simulink library "vmc"  (R2021b)
settings: Solver=VariableStepAuto  StartTime=0.0  StopTime=10.0  RelTol=1e-3
undefined symbols (not defined in the file): AVMC_ACCDeltaTqGradeGn_X_deg, AVMC_ACCDeltaTqIGain4OVRD_X_kph, AVMC_ACCDeltaTqIGain4OVRD_Y_mps2, AVMC_ACCDeltaTqIGain_X_kph, AVMC_ACCDeltaTqIGain_Y_mps2, AVMC_ACCDeltaTqPGain_X_kph, AVMC_ACCDeltaTqPGain_Y_kph, AVMC_ACCGradeofst_X_G, AVMC_ACCGradeofst_Y_pct, AVMC_ACCLoSpdTqLoLim4JP_X_kph, AVMC_ACCLoSpdTqLoLim4JP_Y_deg, AVMC_ACCLoSpdTqLowerLim_X_kph, AVMC_ACCLoSpdTqLowerLim_Y_deg, AVMC_ACCReqAccelGain_X_mps2, AVMC_ACCReqAccelGain_Y_enum, AVMC_ADSPosGFBDeltaTq_X_kph, AVMC_ADSPosGFBDeltaTq_Y_mps2, AVMC_AggressJerkPCT4AT_X_kph, AVMC_AggressJerkPCT_X_kph, AVMC_AggressLimitPCT4AT_X_kph, AVMC_AggressLimitPCT_X_kph, AVMC_DECGradeofst_X_G, AVMC_DECGradeofst_Y_pct, AVMC_DISCDeltaTqIGain_X_kph, AVMC_DISCDeltaTqIGain_Y_mps2, AVMC_DISCDeltaTqPGain_X_kph, AVMC_DISCDeltaTqPGain_Y_kph, AVMC_EPSForceSelect_X_enum, AVMC_EPSForceSelect_Y_enum, AVMC_EPSForceSelectD21_X_enum, AVMC_EPSForceSelectD21_Y_enum, AVMC_ESCRegenOut_X_kph, AVMC_ESCRegenOut_Y_Deg, AVMC_ESCRegenOutEnSpd_X_Deg, AVMC_EstPitchSlopeTs_X_kph, AVMC_GradeCompFlt_X_kph, AVMC_GyroYBandLo_X_Gps, AVMC_HoldResTq_X_kph, AVMC_ISOAccLimit_X_mps, AVMC_ISODecLimit_X_mps, AVMC_ISOJerk_X_mps, AVMC_LatESCRegenOut_X_kph, AVMC_LatESCRegenOut_Y_Deg, AVMC_LongAccDeadZone_X_kph, AVMC_LongAccFiltTsforP2_X_Gps, AVMC_MCPresBaseTq_X_bar, AVMC_MSAPedalOvrd_X_kph, AVMC_MSASpdBand_X_kph, AVMC_MSATqDownEndTq_X_kph, AVMC_MSATqDownTime_X_kph, AVMC_NegZCHoldTq_X_kph, AVMC_OPDDisSlideRate_X_Deg, AVMC_OVRD2ActSR2FCMCMD_X_mps2, AVMC_PedalTqRWhlRatio_X_Nm, AVMC_PedalTqRWhlRatio_Y_gps, AVMC_PedalTqRWhlSlipGain_X_rat, AVMC_PedalTqRWhlSlipGain_Y_kph, AVMC_PedalTqRWhSTRGGain_X_deg, AVMC_PedalTqRWhSTRGGain_Y_kph, AVMC_PosZCHoldTq_X_kph ... (+593)
libraries: hcu_lib x143, simulink x96, tqr x4, $bdroot x1, simulink_extras x1
(part 2 of 17)

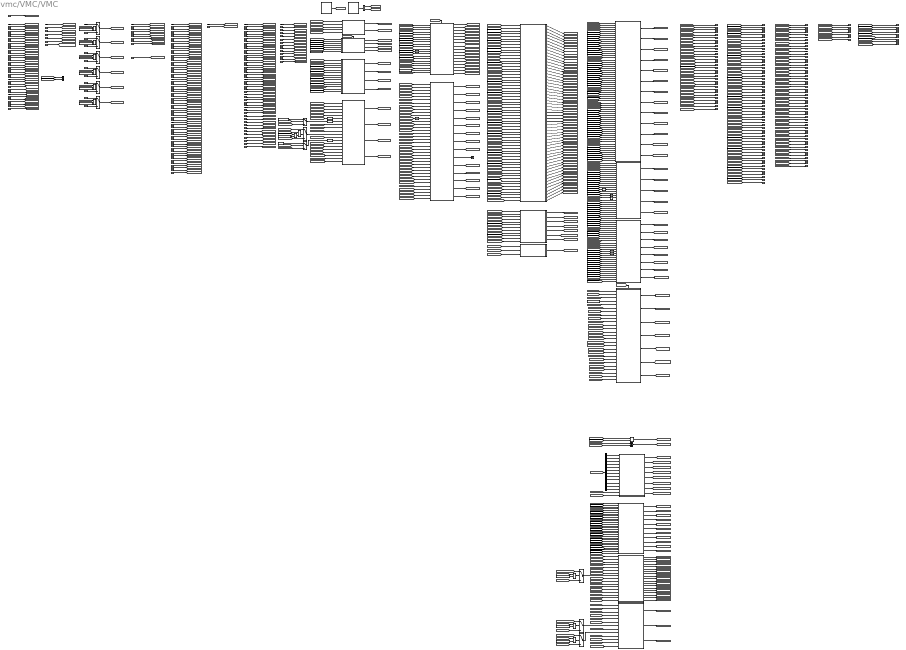
== system vmc/VMC/VMC ==
  note: CAN4
  note: For
      | DDM
      | 2025/02/18
  note: DSC
      | Test
      | Function
  note: SYS
  note: IMU
  note: SafetyControl
  note: ACC_CC_MSAWhlTq
  note: SpeedArbitration
  note: VMC_FCM1
  note: SPD2ACC
  note: PreConditionCheck
  note: KPH2MPH_SetSpeed
  note: CAN1
  note: CAN2
  note: CAN3
  note: DDM
  note: CAN6
  note: GPIO
  note: FD
  note: Phase1_Add Functions for VCU
  note: VMC SW Version:
      | CR-No. B14
      | Date: 2025/07/09
  note: AOICtrl
  task_time_s : Inport
  VINP_DriverSeatBeltCmd_flg : Inport  Port=2
  VINP_MeterIndVehSpeed_kph : Inport  Port=3
  VINP_BrkSwSta_flg : Inport  Port=4
  VINP_EPBSta_enum : Inport  Port=5
  VINP_ACCAvail_flg : Inport  Port=6
  VINP_AEBAvail_flg : Inport  Port=7
  VINP_ESCOFFStatus_enum : Inport  Port=8
  VINP_VehSpeed_kph : Inport  Port=9
  VINP_LFRawWhlSpeed_kph : Inport  Port=10
  VINP_LFRawWhlSpeedV_flg : Inport  Port=11
  VINP_RFRawWhlSpeed_kph : Inport  Port=12
  VINP_RFRawWhlSpeedV_flg : Inport  Port=13
  VINP_LRRawWhlSpeed_kph : Inport  Port=14
  VINP_LRRawWhlSpeedV_flg : Inport  Port=15
  VINP_RRRawWhlSpeed_kph : Inport  Port=16
  VINP_RRRawWhlSpeedV_flg : Inport  Port=17
  VINP_LatAccel_Gps : Inport  Port=18
  VINP_LatAccelV_flg : Inport  Port=19
  VINP_GRADE_Deg : Inport  Port=20
  VINP_LongAccel_Gps : Inport  Port=21
  VINP_MCPressure_bar : Inport  Port=22
  VINP_ESCADASSta_enum : Inport  Port=23
  VINP_FrRBCActive_flg : Inport  Port=24
  VINP_RrRBCActive_flg : Inport  Port=25
  VINP_FrntAxlTrqReqBrk_Nm : Inport  Port=26
  VINP_RearAxlTrqReqBrk_Nm : Inport  Port=27
  VINP_BrkPedalPos_pct : Inport  Port=28
  VINP_SASAngle_Deg : Inport  Port=29
  VINP_ESCActive_flg : Inport  Port=30
  VINP_YawRate_degps : Inport  Port=31
  VINP_RDCActive_enum : Inport  Port=32
  VINP_LFWhlRotDir_enum : Inport  Port=33
  VINP_LRWhlRotDir_enum : Inport  Port=34
  VINP_RFWhlRotDir_enum : Inport  Port=35
  VINP_RRWhlRotDir_enum : Inport  Port=36
  VINP_LongAccelV_flg : Inport  Port=37
  VINP_Distanceunit_flg : Inport  Port=38
  VINP_IVISWCVibModeSta_enum : Inport  Port=39
  VINP_SmartEcoModeSW_flg : Inport  Port=40
  VINP_IVIEPSForceCmd_enum : Inport  Port=41
  VINP_DMSStatus_enum : Inport  Port=42
  VINP_DMSWarningFatigue_enum : Inport  Port=43
  VINP_DMSWarningUnresponsive_flg : Inport  Port=44
  VINP_FrTMSpd_rpm : Inport  Port=45
  VINP_FrTMSpdNidec_rpm : Inport  Port=46
  VINP_RrTMSpd_rpm : Inport  Port=47
  VINP_RrTMSpdNidec_rpm : Inport  Port=48
  VINP_FrEDURealTMTq_Nm : Inport  Port=49
  VINP_FrEDURealTMTqNidec_Nm : Inport  Port=50
  VINP_FrEDURotateDirction_enum : Inport  Port=51
  VINP_FrEDURotateDirctionNidec_enum : Inport  Port=52
  VINP_RrEDURealTMTq_Nm : Inport  Port=53
  VINP_RrEDURealTMTqNidec_Nm : Inport  Port=54
  VINP_RrEDURotateDirction_enum : Inport  Port=55
  VINP_RrEDURotateDirctionNidec_enum : Inport  Port=56
  VINP_ADASAEBSta_enum : Inport  Port=57
  VINP_ADASACCSta_enum : Inport  Port=58
  VINP_ACCRequiredAccel_mps2 : Inport  Port=59
  VINP_ACCVehHoldReq_flg : Inport  Port=60
  VINP_ADASAEBReq_enum : Inport  Port=61
  VINP_ADASLKASta_enum : Inport  Port=62
  VINP_LKAStrToqReq_Nm : Inport  Port=63
  VINP_LKATOIFault_flg : Inport  Port=64
  VINP_LKATOIAct_enum : Inport  Port=65
  VINP_ADASFaultSta_flg : Inport  Port=66
  VINP_AEBVehHoldReq_flg : Inport  Port=67
  VINP_ADASDBSReq_enum : Inport  Port=68
  VINP_ACCObjDist_m : Inport  Port=69
  VINP_ACCObjRelSpd_mps : Inport  Port=70
  VINP_TimeGapLevel_enum : Inport  Port=71
  VINP_HazardWarningReq_flg : Inport  Port=72
  VINP_ADASForceIdle_flg : Inport  Port=73
  VINP_RightTurnLightReq_flg : Inport  Port=74
  VINP_LeftTurnLightReq_flg : Inport  Port=75
  VINP_ForceLowBeam_enum : Inport  Port=76
  VINP_ACCJerkUpperLimit_mps3 : Inport  Port=77
  VINP_ACCComfortBandUpper_mps2 : Inport  Port=78
  VINP_ACCJerkLowerLimit_mps3 : Inport  Port=79
  VINP_ACCComfortBandLower_mps2 : Inport  Port=80
  VINP_ADASVehSpdLim_raw32 : Inport  Port=81
  VINP_ADASShftPosnReqA_flg : Inport  Port=82
  VINP_ADASShftPosnReq_enum : Inport  Port=83
  VINP_ADASFCWSta_enum : Inport  Port=84
  VINP_ADASLDWSta_enum : Inport  Port=85
  VINP_ADASFltWrnReq_flg : Inport  Port=86
  VINP_ACCObjDstLvl_enum : Inport  Port=87
  VINP_ACCTakeoverReq_flg : Inport  Port=88
  VINP_ADASWarningMsg_enum : Inport  Port=89
  VINP_ADASCAMSpdLim_enum : Inport  Port=90
  VINP_TargetType_enum : Inport  Port=91
  VINP_ADASSLIFSpdLim_enum : Inport  Port=92
  VINP_LKAHODDisplayWarning_flg : Inport  Port=93
  VINP_LKAHODSoundWarning_flg : Inport  Port=94
  VINP_ADASLFCSta_enum : Inport  Port=95
  VINP_ADASLaneModeL_enum : Inport  Port=96
  VINP_ADASLaneModeR_enum : Inport  Port=97
  VINP_ADASSLIFSta_enum : Inport  Port=98
  VINP_ADASISASta_enum : Inport  Port=99
  VINP_ADASLDWMute_flg : Inport  Port=100
  VINP_ADASFCWMute_flg : Inport  Port=101
  VINP_ADASLFCHandsOffWarning_enum : Inport  Port=102
  VINP_LVDADisabled_flg : Inport  Port=103
  VINP_LVDAMuteSta_enum : Inport  Port=104
  VINP_LVDAFailinfo_flg : Inport  Port=105
  VINP_LVDAWarning_flg : Inport  Port=106
  VINP_LVDAACCStatusInformation_flg : Inport  Port=107
  VINP_ADASLFCWarnSound_enum : Inport  Port=108
  VINP_FCMACCmode_enum : Inport  Port=109
  VINP_ADASLanetypeR_enum : Inport  Port=110
  VINP_ADASLanetypeL_enum : Inport  Port=111
  VINP_ADASLanecurveL_raw32 : Inport  Port=112
  VINP_ADASLanecurveR_raw32 : Inport  Port=113
  VINP_ADASDrvInputTqBoostAct_flg : Inport  Port=114
  VINP_ADASStrWhlAngCtrlStatus_flg : Inport  Port=115
  VINP_ADASMaxAngCtrlOutTqLimit_Nm : Inport  Port=116
  VINP_ADASDrvInputTqBoostGain_pct : Inport  Port=117
  VINP_ADASAngCtrlTqWeightGain_pct : Inport  Port=118
  VINP_ADASDesStrWhlAngCtrlCmd_Deg : Inport  Port=119
  VINP_BrakeSWGPIO_flg : Inport  Port=120
  VINP_HoodSW_flg : Inport  Port=121
  APP_SpdLimit_flg : Inport  Port=122
  APP_SpdLimit : Inport  Port=123
  VINP_DIDGetDynoMode_flg : Inport  Port=124
  VINP_VehicleType_enum : Inport  Port=125
  VINP_SWCType_enum : Inport  Port=126
  VINP_APSStaSystem_enum : Inport  Port=127
  VINP_APSDecReqA_flg : Inport  Port=128
  VINP_APSDecReq_mps2 : Inport  Port=129
  VINP_APSReq_enum : Inport  Port=130
  VINP_APSShiftPosnReq_enum : Inport  Port=131
  VINP_APSSpeedCMD_kph : Inport  Port=132
  VINP_APSVMCReqA_flg : Inport  Port=133
  VINP_CAASVMCReqA_flg : Inport  Port=134
  VINP_APSVRqEPASCtrl_flg : Inport  Port=135
  VINP_APSRqEPASCtrl_flg : Inport  Port=136
  VINP_APSAngleTarget_Deg : Inport  Port=137
  VBCM_DrDoorSW_flg : Inport  Port=138
  VDSC_DISCTurn_flg : Inport  Port=139
  VDSC_DISCSta_enum : Inport  Port=140
  VDSC_DISCTargetSpd_kph : Inport  Port=141
  VDSC_TurningSpdMovingflat_kph : Inport  Port=142
  VDSC_AutoTurnMode_flg : Inport  Port=143
  VDSC_AccDecResp_flg : Inport  Port=144
  VDSC_PreACC_flg : Inport  Port=145
  VDSC_PreACC_mps2 : Inport  Port=146
  VTQD_DriverWhlTqDem_Nm : Inport  Port=147
  VTQD_CoordWhlTqDemFr_Nm : Inport  Port=148
  VTQD_CoordWhlTqDemRr_Nm : Inport  Port=149
  VTQD_GearActualPosn_enum : Inport  Port=150
  VTQD_ExternalTqAllow_flg : Inport  Port=151
  VTQD_LowIdleAccPedal_flg : Inport  Port=152
  VTQD_ExtShftAllow_flg : Inport  Port=153
  VTQD_FrEDUAvailBrkRgnTq_Nm : Inport  Port=154
  VTQD_RrEDUAvailBrkRgnTq_Nm : Inport  Port=155
  VTQD_APSStaSys_enum : Inport  Port=156
  VTQD_APSDecReqA_flg : Inport  Port=157
  VTQD_APSDecReq_mps2 : Inport  Port=158
  VTQD_APSReq_enum : Inport  Port=159
  VTQD_AfterAvailableTqDemFr_Nm : Inport  Port=160
  VTQD_AfterAvailableTqDemRr_Nm : Inport  Port=161
  VTQD_EquivAccPedalSWSta_flg : Inport  Port=162
  VTQD_ExtDoorAllow_flg : Inport  Port=163
  VTQD_SpdCtrlSta_flg : Inport  Port=164
  VTQD_SpdCtrlMode_enum : Inport  Port=165
  VTQD_RegenMode_enum : Inport  Port=166
  VTQD_SetSpd_kph : Inport  Port=167
  VTQD_SWC2ResUpSta_flg : Inport  Port=168
  VTQD_SWC2SetdownSta_flg : Inport  Port=169
  VTQD_SWC2CANCELSta_flg : Inport  Port=170
  VTQD_CreepBaseTqD_Nm : Inport  Port=171
  VTQD_VehActSpd_kph : Inport  Port=172
  VTQD_EVDriveMode_enum : Inport  Port=173
  VTQD_SWC1CANCELSta_flg : Inport  Port=174
  VTQD_SWC1ResUpSta_flg : Inport  Port=175
  VTQD_SWC1SetdownSta_flg : Inport  Port=176
  VTQD_PreLoadPreEn_flg : Inport  Port=177
  VTQD_EPBCarWashMode_flg : Inport  Port=178
  VTQR_RrTMTqReq_Nm : Inport  Port=179
  VTQR_FrTMTqReq_Nm : Inport  Port=180
  VDHP_ActAPSPosn_pct : Inport  Port=181
  <VPMM_DrivetrainSelect_enum> : Inport  Port=182
  BINP_IMU_outputs : Inport  Port=183  OutDataTypeStr=Bus: BINP_IMU_outputs
  VDDM_VMCLongCtrlProhibited_flg : Inport  Port=184
  VDDM_VMCLatCtrlProhibited_flg : Inport  Port=185
  VDDM_ESC1Err_flg : Inport  Port=186
  VDDM_ESC5Err_flg : Inport  Port=187
  VDDM_VMCEPSErr_flg : Inport  Port=188
  VDDM_VCURAPSErrLv2_flg : Inport  Port=189
  VDDM_VCURAPSErrLv3_flg : Inport  Port=190
  VDDM_LimpHomeAct_flg : Inport  Port=191
  VDDM_VCUMSAErr_flg : Inport  Port=192
  VINP_SCPSystemMode_enum : Inport  Port=193
  ACC_Function : Subsystem
  AND{4..6,9} (4 alike) : Logic  AllPortsSameDT=off  OutDataTypeStr=boolean
  APS function : Subsystem
  Add : Sum
  Bus Selector10 : BusSelector  OutputSignals=VINP_MemOffsetGyroX_raw16,VINP_MemOffsetGyroY_raw16,VINP_MemOffsetGyroZ_raw16,VINP_MemOffsetAccX_raw16,VINP_MemOffsetAccY_raw16,VINP_MemOffsetAccZ_raw16,VINP_SensingGyroX_raw16,VINP_SensingGyroY_raw16,VINP_SensingGyroZ_raw16,VINP_SensingAccX_raw16,VINP_SensingAccY_raw16,VINP_SensingAccZ_raw16
  Cast To Single{7,31,33..34} (4 alike) : DataTypeConversion  OutDataTypeStr=uint8
  Constant1 : Constant  Value=C_TASK_10MS_S
  Constant10 : Constant  Value=KVMC_RDCRzSource_flg
  Constant109 : Constant  Value=TRUE
  Constant11 : Constant  Value=KVMC_SlideRateGxSource_flg
  Constant{3..6,8,14} (6 alike) : Constant  Value=ENUM_VEHICLETYPE_D31L24
  Constant15 : Constant  Value=ENUM_DISCSTA_ACTIVE
  Constant2 : Constant  Value=C_TASK_10MS_S
  Constant26 : Constant  Value=C_TASK_10MS_S
  Constant28 : Constant  Value=KVMC_RDCGySource_flg
  Constant7 : Constant  Value=ENUM_DISCSTA_ACTIVE
  CruiseControlFunction : Subsystem
  EPSForceSelect : Subsystem
  Equal{1..6} (6 alike) : RelationalOperator  Operator=~=  OutDataTypeStr=boolean  RndMeth=Simplest
  FeatureSetSpeed : Subsystem
  Function-Call Split : FunctionCallSplit  IconShape=distinctive  NumOutputPorts=2  OutputPortLayout=default
  IMU : Subsystem
  LFCAOIControl : Subsystem
  Logical Operator : Logic  Operator=OR  AllPortsSameDT=off  OutDataTypeStr=boolean
  Long Acceleration Calculation : Subsystem  TreatAsAtomicUnit=on
  MSA function : Subsystem
  PreConditionCheck : Subsystem
  RDC Determination : Subsystem
  Relational Operator8 : RelationalOperator  Operator=~=  OutDataTypeStr=boolean  RndMeth=Simplest
  SPD2ACC : Subsystem
  SafetyControl : Subsystem  TreatAsAtomicUnit=on
  Scheduler : Stateflow chart  TreatAsAtomicUnit=on
  Scheduler1 : Stateflow chart  TreatAsAtomicUnit=on
  Slide Rate  Calculation : Subsystem
  SpeedArbitration : Subsystem
  SpeedCalculation : Subsystem  TreatAsAtomicUnit=on
  Switch{1..12} (12 alike) : Switch  Criteria=u2 > Threshold
  Terminator : Terminator
  Terminator1 : Terminator
  Terminator2 : Terminator
  Unit Delay{1,5..8} (5 alike) : UnitDelay  SampleTime=-1  HasFrameUpgradeWarning=on
  VMC_FCM1 : Subsystem
  initial = 0 : UnitDelay  SampleTime=-1  HasFrameUpgradeWarning=on
  VVMC_FeatSetSpdFinal_raw32 : Outport
  VVMC_VehicleSpeed_mph : Outport  Port=2
  VVMC_VehicleSpeed_kph : Outport  Port=3
  VVMC_MeterIndSpeed_raw32 : Outport  Port=4
  VVMC_MeterIndSpeedForCalcu_kph : Outport  Port=5
  VVMC_VMCAEBCtrlAvail_flg : Outport  Port=6
  VVMC_VMCACCCtrlAvail_flg : Outport  Port=7
  VVMC_VMCCCCtrlAvail_flg : Outport  Port=8
  VVMC_VMCMSACtrlAvail_flg : Outport  Port=9
  VVMC_FeatArbitrSta_enum : Outport  Port=10
  VVMC_FeatReqSpd_kph : Outport  Port=11
  VVMC_JerkPCT_pct : Outport  Port=12
  VVMC_LimitPCT_pct : Outport  Port=13
  VVMC_LFWhlSpeedRollAve_kph : Outport  Port=14
  VVMC_RFWhlSpeedRollAve_kph : Outport  Port=15
  VVMC_LRWhlSpeedRollAve_kph : Outport  Port=16
  VVMC_RRWhlSpeedRollAve_kph : Outport  Port=17
  VVMC_FrontRearSlipRatioCtrl_flg : Outport  Port=18
  VVMC_RearWhlSlipRatioCtrl_flg : Outport  Port=19
  VVMC_SingleWhlSlipRatioCtrl_flg : Outport  Port=20
  VVMC_LatAccCtrl_flg : Outport  Port=21
  VVMC_SafetyCtrl_flg : Outport  Port=22
  VVMC_EstSlope_Deg : Outport  Port=23
  VVMC_SPD2ACCAct_flg : Outport  Port=24
  VVMC_AccCalcuPID_mps2 : Outport  Port=25
  VVMC_ISOAccLimit_mps2 : Outport  Port=26
  VVMC_ISODecLimit_mps2 : Outport  Port=27
  VVMC_ISOJerkLimit_mps3 : Outport  Port=28
  VVMC_ACCRequiredAccel_mps2 : Outport  Port=29
  VVMC_DISCReqAcc_mps2 : Outport  Port=30
  VVMC_FeatArbitrFinal_enum : Outport  Port=31
  VVMC_ActACCRequiredAccel_mps2 : Outport  Port=32
  VVMC_LateralCtrl_flg : Outport  Port=33
  VVMC_ADASLKASta_enum : Outport  Port=34
  VVMC_LKAStrToqReq_Nm : Outport  Port=35
  VVMC_LKATOIFault_flg : Outport  Port=36
  VVMC_LKATOIAct_enum : Outport  Port=37
  VVMC_ADASAEBReq_enum : Outport  Port=38
  VVMC_ADASFaultSta_flg : Outport  Port=39
  VVMC_AEBVehHoldReq_flg : Outport  Port=40
  VVMC_ACCVehHoldReq_flg : Outport  Port=41
  VVMC_ADASDBSReq_enum : Outport  Port=42
  VVMC_ADASACCSta_enum : Outport  Port=43
  VVMC_ACCObjDist_m : Outport  Port=44
  VVMC_ACCObjRelSpd_mps : Outport  Port=45
  VVMC_TimeGapLevel_enum : Outport  Port=46
  VVMC_ACCJerkUpperLimit_mps3 : Outport  Port=47
  VVMC_ACCComfortBandUpper_mps2 : Outport  Port=48
  VVMC_ACCJerkLowerLimit_mps3 : Outport  Port=49
  VVMC_ACCComfortBandLower_mps2 : Outport  Port=50
  VVMC_ADASVehSpdLim_raw32 : Outport  Port=51
  VVMC_ADASShftPosnReqA_flg : Outport  Port=52
  VVMC_ADASShftPosnReq_enum : Outport  Port=53
  VVMC_ADASForceIdle_flg : Outport  Port=54
  VVMC_HazardWarningReq_flg : Outport  Port=55
  VVMC_RightTurnLightReq_flg : Outport  Port=56
  VVMC_LeftTurnLightReq_flg : Outport  Port=57
  VVMC_ADASFCWSta_enum : Outport  Port=58
  VVMC_ADASLDWSta_enum : Outport  Port=59
  VVMC_ADASFltWrnReq_flg : Outport  Port=60
  VVMC_ACCObjDstLvl_enum : Outport  Port=61
  VVMC_ForceLowBeam_enum : Outport  Port=62
  VVMC_ACCTakeoverReq_flg : Outport  Port=63
  VVMC_ADASWarningMsg_enum : Outport  Port=64
  VVMC_ADASCAMSpdLim_enum : Outport  Port=65
  VVMC_TargetType_enum : Outport  Port=66
  VVMC_ADASSLIFSpdLim_enum : Outport  Port=67
  VVMC_LKAHODDisplayWarning_flg : Outport  Port=68
  VVMC_LKAHODSoundWarning_flg : Outport  Port=69
  VVMC_ADASLFCSta_enum : Outport  Port=70
  VVMC_ADASLaneModeL_enum : Outport  Port=71
  VVMC_ADASLaneModeR_enum : Outport  Port=72
  VVMC_ADASSLIFSta_enum : Outport  Port=73
  VVMC_ADASISASta_enum : Outport  Port=74
  VVMC_ADASLDWMute_flg : Outport  Port=75
  VVMC_ADASFCWMute_flg : Outport  Port=76
  VVMC_ADASLFCHandsOffWarning_enum : Outport  Port=77
  VVMC_LVDADisabled_flg : Outport  Port=78
  VVMC_LVDAMuteSta_enum : Outport  Port=79
  VVMC_LVDAFailinfo_flg : Outport  Port=80
  VVMC_LVDAWarning_flg : Outport  Port=81
  VVMC_LVDAACCStatusInformation_flg : Outport  Port=82
  VVMC_ADASLFCWarnSound_enum : Outport  Port=83
  VVMC_FCMACCmode_enum : Outport  Port=84
  VVMC_ADASLanetypeR_enum : Outport  Port=85
  VVMC_ADASLanetypeL_enum : Outport  Port=86
  VVMC_ADASLanecurveL_raw32 : Outport  Port=87
  VVMC_ADASLanecurveR_raw32 : Outport  Port=88
  VVMC_ADASAEBSta_enum : Outport  Port=89
  VVMC_FCMLDWRequest_enum : Outport  Port=90
  VVMC_FCMLDWFault_flg : Outport  Port=91
  VVMC_ADASActive_flg : Outport  Port=92
  VVMC_ACCCtrlAvail_flg : Outport  Port=93
  VVMC_ADASNegReq_flg : Outport  Port=94
  VVMC_ACCPedalOvrd_flg : Outport  Port=95
  VVMC_ADASWhlTqReq_Nm : Outport  Port=96
  VVMC_AccPedalOvrdDISC_flg : Outport  Port=97
  VVMC_RearTqRatio_rat : Outport  Port=98
  VVMC_TimeGapCalcu_s : Outport  Port=99
  VVMC_CCCtrlSta_enum : Outport  Port=100
  VVMC_CruzActive_flg : Outport  Port=101
  VVMC_CCPedalOvrd_flg : Outport  Port=102
  VVMC_CruzWhlTqReq_Nm : Outport  Port=103
  VVMC_MSACtrlSta_enum : Outport  Port=104
  VVMC_MSAActive_flg : Outport  Port=105
  VVMC_MSAWhlTqReq_Nm : Outport  Port=106
  VVMC_APSCtrlAvail_flg : Outport  Port=107
  VVMC_APSActive_flg : Outport  Port=108
  VVMC_APSSpeedCMD_kph : Outport  Port=109
  VVMC_APSShiftPosnReq_enum : Outport  Port=110
  VVMC_APSStaSys_enum : Outport  Port=111
  VVMC_APSDecReqA_flg : Outport  Port=112
  VVMC_APSDecReq_mps2 : Outport  Port=113
  VVMC_APSReq_enum : Outport  Port=114
  VVMC_LongAcc_Gps : Outport  Port=115
  VVMC_RawWhlSpdSlideRate_pct : Outport  Port=116
  VVMC_LFWhlSpdSlideRate_pct : Outport  Port=117
  VVMC_RFWhlSpdSlideRate_pct : Outport  Port=118
  VVMC_LRWhlSpdSlideRate_pct : Outport  Port=119
  VVMC_RRWhlSpdSlideRate_pct : Outport  Port=120
  VVMC_PredictVehSpd_kph : Outport  Port=121
  VVMC_LF4WhlSpdSlideRate_pct : Outport  Port=122
  VVMC_RF4WhlSpdSlideRate_pct : Outport  Port=123
  VVMC_LR4WhlSpdSlideRate_pct : Outport  Port=124
  VVMC_RR4WhlSpdSlideRate_pct : Outport  Port=125
  VVMC_4WhlSpdSlideRate_pct : Outport  Port=126
  VVMC_ActMaxSlideRate_pct : Outport  Port=127
  VVMC_ActLFSlideRate_pct : Outport  Port=128
  VVMC_ActRFSlideRate_pct : Outport  Port=129
  VVMC_ActLRSlideRate_pct : Outport  Port=130
  VVMC_ActRRSlideRate_pct : Outport  Port=131
  VVMC_AltLWhlSlideRate_pct : Outport  Port=132
  VVMC_AltRWhlSlideRate_pct : Outport  Port=133
  VVMC_AltWhlSlideRate_pct : Outport  Port=134
  VVMC_CCMSASpdWar_flg : Outport  Port=135
  VVMC_IMUEnaCmd_flg : Outport  Port=136
  VVMC_RWDRDCActive_enum : Outport  Port=137
  VVMC_MSAWhlTqActive_flg : Outport  Port=138
  VVMC_RDCEnSlideRate_pct : Outport  Port=139
  VVMC_ActStESCYaw_Dps : Outport  Port=140
  VVMC_ACCOvrdMemTq_Nm : Outport  Port=141
  VVMC_CAASCtrlAvail_flg : Outport  Port=142
  VVMC_CAASActive_flg : Outport  Port=143
  "VVMC_ExtraMSACtrlSta_enum " : Outport  Port=144
  VVMC_CalibratedAccX_G : Outport  Port=145
  VVMC_CalibratedAccY_G : Outport  Port=146
  VVMC_CalibratedAccZ_G : Outport  Port=147
  VVMC_CalibratedGyroX_Dps : Outport  Port=148
  VVMC_CalibratedGyroY_Dps : Outport  Port=149
  VVMC_CalibratedGyroZ_Dps : Outport  Port=150
  VVMC_SetACCDisableAPS_flg : Outport  Port=151
  VVMC_FDCVMCAPSVRqEPSCtrl_flg : Outport  Port=152
  VVMC_FDCVMCAPSAngleTarget_deg : Outport  Port=153
  VVMC_FDCVMCAPSRqEPSCtrl_flg : Outport  Port=154
  VVMC_FDCVMCAngCtrlTqWtGn_pct : Outport  Port=155
  VVMC_FDCVMCDrInpTqBstAct_flg : Outport  Port=156
  VVMC_FDCVMCMaxAngCtrlOutTqLim_Nm : Outport  Port=157
  VVMC_FDCVMCDrInpTqBstGn_pct : Outport  Port=158
  VVMC_VehPitchAngleSta_enum : Outport  Port=159
  VVMC_DMSModeCmd_enum : Outport  Port=160
  wires:
  [VVMC_DMSModeCmd_enum] -> VVMC_DMSModeCmd_enum/1
  EPSForceSelect/1(VVMC_DMSModeCmd_enum) -> [VVMC_DMSModeCmd_enum]
  [VINP_VehicleType_enum] -> EPSForceSelect/3(VINP_VehicleType_enum)
  [VPMM_DrivetrainSelect_enum] -> EPSForceSelect/2(VPMM_DrivetrainSelect_enum)
  [VINP_IVIEPSForceCmd_enum] -> EPSForceSelect/1(VINP_IVIEPSForceCmd_enum)
  VINP_IVIEPSForceCmd_enum/1 -> [VINP_IVIEPSForceCmd_enum]
  [VPMM_DrivetrainSelect_enum] -> RDC Determination/13(VPMM_DrivetrainSelect_enum)
  [VINP_VehicleType_enum] -> RDC Determination/12(VINP_VehicleType_enum)
  [VTQD_ExtDoorAllow_flg] -> SafetyControl/21(VTQD_ExtDoorAllow_flg)
  SafetyControl/13(VVMC_VehPitchAngleSta_enum) -> [VVMC_VehPitchAngleSta_enum]
  Constant2/1 -> SafetyControl/20(task_time_s)
  [VVMC_CalibratedAccXAftRA_G] -> SafetyControl/19(VVMC_CalibratedAccXAftRA_G)
  IMU/8(VVMC_CalibratedAccXAftRA_G) -> [VVMC_CalibratedAccXAftRA_G]
  [VINP_VehicleType_enum] -> IMU/14(VINP_VehicleType_enum)
  [VPMM_DrivetrainSelect_enum] -> SPD2ACC/34(VPMM_DrivetrainSelect_enum)
  [VINP_RearAxlTrqReqBrk_Nm] -> SPD2ACC/33(VINP_RearAxlTrqReqBrk_Nm)
  [VINP_FrntAxlTrqReqBrk_Nm] -> SPD2ACC/32(VINP_FrntAxlTrqReqBrk_Nm)
  ACC_Function/11(VVMC_ACCCtrlAllow_flg) -> [VVMC_ACCCtrlAllow_flg]
  [VVMC_VMCACCCtrlAvail_flg] -> ACC_Function/52(VVMC_VMCACCCtrlAvail_flg)
  [VINP_LongAccelV_flg] -> Long Acceleration Calculation/9(VINP_LongAccelV_flg)
  [VDDM_ESC5Err_flg] -> Long Acceleration Calculation/8(VDDM_ESC5Err_flg)
  [VDDM_VCUMSAErr_flg] -> PreConditionCheck/14(VDDM_VCUMSAErr_flg)
  [VDDM_LimpHomeAct_flg] -> PreConditionCheck/13(VDDM_LimpHomeAct_flg)
  VDDM_VCUMSAErr_flg/1 -> [VDDM_VCUMSAErr_flg]
  VDDM_LimpHomeAct_flg/1 -> [VDDM_LimpHomeAct_flg]
  [VINP_SWCType_enum] -> ACC_Function/51(VINP_SWCType_enum)
  [VTQD_SWC1ResUpSta_flg] -> ACC_Function/50(VTQD_SWC1ResUpSta_flg)
  VDDM_VCURAPSErrLv3_flg/1 -> [VDDM_VCURAPSErrLv3_flg]
  VDDM_VCURAPSErrLv2_flg/1 -> [VDDM_VCURAPSErrLv2_flg]
  VTQD_EPBCarWashMode_flg/1 -> [VTQD_EPBCarWashMode_flg]
  VINP_SCPSystemMode_enum/1 -> [VINP_SCPSystemMode_enum]
  [VTQD_APSStaSys_enum] -> APS function/11(VTQD_APSStaSys_enum)
  [VINP_APSReq_enum] -> APS function/18(VINP_APSReq_enum)
  [VINP_ADASACCSta_enum] -> APS function/22(VINP_ADASACCSta_enum)
  [VINP_APSStaSystem_enum] -> APS function/15(VINP_APSStaSystem_enum)
  [VINP_APSDecReqA_flg] -> APS function/16(VINP_APSDecReqA_flg)
  [VTQD_ExtShftAllow_flg] -> APS function/2(VTQD_ExtShiftAllow_flg)  "VTQD_ExtShftAllow_flg"
  [VINP_BrkPedalPos_pct] -> APS function/25(VINP_BrkPedalPos_pct)
  [VINP_BrkSwSta_flg] -> APS function/23(VINP_BrkSwSta_flg)
  [task_time_s] -> APS function/8(task_time_s)  "task_time_s"
  [VINP_MCPressure_bar] -> APS function/24(VINP_MCPressure_bar)
  [VTQD_GearActualPosn_enum] -> APS function/4(VTQD_GearActualPosn_enum)  "VAPS_APSStaSystem_enum"
  [VDDM_VCURAPSErrLv3_flg] -> APS function/29(VDDM_VCURAPSErrLv3_flg)
  [VVMC_CruzActive_flg] -> APS function/20(VVMC_CruzActive_flg)
  [VVMC_MeterIndSpeedForCalcu_kph] -> APS function/27(VVMC_MeterIndSpeedForCalcu_kph)
  [VVMC_VehicleSpeed_kph] -> APS function/19(VVMC_VehicleSpeed_kph)
  [VTQD_ExtDoorAllow_flg] -> APS function/3(VTQD_ExtDoorAllow_flg)
  [VTQD_EPBCarWashMode_flg] -> APS function/30(VTQD_EPBCarWashMode_flg)
  [VINP_ACCObjDist_m] -> APS function/26(VINP_ACCObjDist_m)
  [VDDM_VCURAPSErrLv2_flg] -> APS function/28(VDDM_VCURAPSErrLv2_flg)
  [VINP_APSDecReq_mps2] -> APS function/17(VINP_APSDecReq_mps2)
  [VINP_CAASVMCReqA_flg] -> APS function/21(VINP_CAASVMCReqA_flg)
  [VINP_APSShiftPosnReq_enum] -> APS function/6(VINP_APSShiftPosnReq_enum)  "VAPS_APSShiftPosnReq_enum"
  [VTQD_APSDecReq_mps2] -> APS function/13(VTQD_APSDecReq_mps2)
  [VVMC_ADASActive_flg] -> APS function/10(VVMC_ADASActive_flg)
  [VINP_APSSpeedCMD_kph] -> APS function/7(VINP_APSSpeedCMD_kph)  "VAPS_APSSpeedCMD_kph"
  [VTQD_APSDecReqA_flg] -> APS function/12(VTQD_APSDecReqA_flg)
  [VINP_APSVMCReqA_flg] -> APS function/5(VINP_APSVMCReqA_flg)  "VAPS_APSVMCReqA_flg"
  [VTQD_ExternalTqAllow_flg] -> APS function/1(VTQD_ExternalTqAllow_flg)  "VTQD_ExternalTqAllow_flg"
  [VINP_SCPSystemMode_enum] -> APS function/9(VINP_SCPSystemMode_enum)
  [VTQD_APSReq_enum] -> APS function/14(VTQD_APSReq_enum)
  [VVMC_FeatSetSpdFinal_raw32] -> MSA function/29(VVMC_FeatSetSpdFinal_raw32)
  [VVMC_FeatSetSpdFinal_raw32] -> CruiseControlFunction/26(VVMC_FeatSetSpdFinal_raw32)
  [VINP_ACCRequiredAccel_mps2] -> ACC_Function/49(VINP_ACCRequiredAccel_mps2)  "VINP_ACCRequiredAccel_mps2"
  [VVMC_OVRD2ActRampActive_flg] -> ACC_Function/48(VVMC_OVRD2ActRampActive_flg)
  SPD2ACC/14(VVMC_OVRD2ActRampActive_flg) -> [VVMC_OVRD2ActRampActive_flg]
  [VDDM_VMCEPSErr_flg] -> LFCAOIControl/12(VDDM_VMCEPSErr_flg)
  [VVMC_VehicleSpeed_kph] -> SafetyControl/1(VVMC_VehicleSpeed_kph)
  [VINP_GRADE_Deg] -> SafetyControl/14(VINP_GRADE_deg)
  [VINP_LongAccel_Gps] -> SafetyControl/13(VINP_LongAccel_Gps)
  [VINP_LatAccelV_flg] -> SafetyControl/11(VINP_LatAccelV_flg)
  [VINP_LatAccel_Gps] -> SafetyControl/10(VINP_LatAccel_Gps)
  [VINP_RRRawWhlSpeedV_flg] -> SafetyControl/9(VINP_RRRawWhlSpeedV_flg)
  [VINP_RRRawWhlSpeed_kph] -> SafetyControl/8(VINP_RRRawWhlSpeed_kph)
  [VINP_LRRawWhlSpeedV_flg] -> SafetyControl/7(VINP_LRRawWhlSpeedV_flg)
  [VINP_LRRawWhlSpeed_kph] -> SafetyControl/6(VINP_LRRawWhlSpeed_kph)
  [VINP_RFRawWhlSpeedV_flg] -> SafetyControl/5(VINP_RFRawWhlSpeedV_flg)
  [VINP_RFRawWhlSpeed_kph] -> SafetyControl/4(VINP_RFRawWhlSpeed_kph)
  [VINP_LFRawWhlSpeedV_flg] -> SafetyControl/3(VINP_LFRawWhlSpeedV_flg)
  [VINP_LFRawWhlSpeed_kph] -> SafetyControl/2(VINP_LFRawWhlSpeed_kph)
  [VVMC_IMUEnaCmd_flg] -> SafetyControl/16(VVMC_IMUEnaCmd_flg)
  [VVMC_CalibratedAccX_G] -> SafetyControl/15(VVMC_CalibratedAccX_G)
  [VDDM_ESC5Err_flg] -> SafetyControl/18(VDDM_ESC5Err_flg)
  [VDDM_ESC1Err_flg] -> SafetyControl/17(VDDM_ESC1Err_flg)
  initial = 0/1 -> SafetyControl/12(VVMC_FeatArbitrFinal_enum)  "VVMC_FeatArbitrFinal_enum"
  SafetyControl/12(VVMC_FrRrSlipSpd_kph) -> [VVMC_FrRrSlipSpd_kph]
  SafetyControl/11(VVMC_LongAccelCalcuByVehSpdRaw_gps) -> [VVMC_LongAccelCalcuByVehSpdRaw_gps]
  SafetyControl/10(VVMC_RRWhlSpeedRollAve_kph) -> [VVMC_RRWhlSpeedRollAve_kph]
  SafetyControl/9(VVMC_LRWhlSpeedRollAve_kph) -> [VVMC_LRWhlSpeedRollAve_kph]
  SafetyControl/8(VVMC_RFWhlSpeedRollAve_kph) -> [VVMC_RFWhlSpeedRollAve_kph]
  SafetyControl/7(VVMC_LFWhlSpeedRollAve_kph) -> [VVMC_LFWhlSpeedRollAve_kph]
  SafetyControl/6(VVMC_EstSlope_Deg) -> [VVMC_EstSlopeCal_Deg]
  SafetyControl/5(VVMC_LatAccCtrl_flg) -> [VVMC_LatAccCtrl_flg]
  SafetyControl/4(VVMC_SingleWhlSlipRatioCtrl_flg) -> [VVMC_SingleWhlSlipRatioCtrl_flg]
  SafetyControl/3(VVMC_RearWhlSlipRatioCtrl_flg) -> [VVMC_RearWhlSlipRatioCtrl_flg]
  SafetyControl/1(VVMC_SafetyCtrl_flg) -> [VVMC_SafetyCtrl_flg]
  SafetyControl/2(VVMC_FrontRearSlipRatioCtrl_flg) -> [VVMC_FrontRearSlipRatioCtrl_flg]
  [VTQD_VehActSpd_kph] -> SpeedCalculation/4(VTQD_VehActSpd_kph)
  [VINP_Distanceunit_flg] -> SpeedCalculation/2(VINP_Distanceunit_flg)  "VINP_Distanceunit_flg"
  [VDDM_ESC5Err_flg] -> SpeedCalculation/6(VDDM_ESC5Err_flg)
  [VDDM_ESC1Err_flg] -> SpeedCalculation/5(VDDM_ESC1Err_flg)
  [VINP_VehSpeed_kph] -> SpeedCalculation/3(VINP_VehSpeed_kph)
  [VINP_MeterIndVehSpeed_kph] -> SpeedCalculation/1(VINP_MeterIndVehSpeed_kph)  "VINP_METERKPHCalcu_kph"
  [VDDM_VMCLatCtrlProhibited_flg] -> LFCAOIControl/11(VDDM_VMCLatCtrlProhibited_flg)
  [VDDM_VMCLongCtrlProhibited_flg] -> VMC_FCM1/61(VDDM_VMCLongCtrlProhibited_flg)
  [VDDM_VMCLatCtrlProhibited_flg] -> VMC_FCM1/60(VDDM_VMCLatCtrlProhibited_flg)
  [VINP_IVISWCVibModeSta_enum] -> VMC_FCM1/59(VINP_IVISWCVibModeSta_enum)
  [VDDM_VMCLongCtrlProhibited_flg] -> PreConditionCheck/12(VDDM_VMCLongCtrlProhibited_flg)
  VDDM_VMCLongCtrlProhibited_flg/1 -> [VDDM_VMCLongCtrlProhibited_flg]
  VDDM_VMCLatCtrlProhibited_flg/1 -> [VDDM_VMCLatCtrlProhibited_flg]
  VDDM_ESC1Err_flg/1 -> [VDDM_ESC1Err_flg]
  VDDM_ESC5Err_flg/1 -> [VDDM_ESC5Err_flg]
  VDDM_VMCEPSErr_flg/1 -> [VDDM_VMCEPSErr_flg]
  LFCAOIControl/7(VVMC_FDCVMCDrInpTqBstGn_pct) -> [VVMC_FDCVMCDrInpTqBstGn_pct]
  LFCAOIControl/5(VVMC_FDCVMCDrInpTqBstAct_flg) -> [VVMC_FDCVMCDrInpTqBstAct_flg]
  LFCAOIControl/4(VVMC_FDCVMCAngCtrlTqWtGn_pct) -> [VVMC_FDCVMCAngCtrlTqWtGn_pct]
  LFCAOIControl/3(VVMC_FDCVMCAPSAngleTarget_deg) -> [VVMC_FDCVMCAPSAngleTarget_deg]
  LFCAOIControl/2(VVMC_FDCVMCAPSRqEPSCtrl_flg) -> [VVMC_FDCVMCAPSRqEPSCtrl_flg]
  LFCAOIControl/1(VVMC_FDCVMCAPSVRqEPSCtrl_flg) -> [VVMC_FDCVMCAPSVRqEPSCtrl_flg]
  LFCAOIControl/6(VVMC_FDCVMCMaxAngCtrlOutTqLim_Nm) -> [VVMC_FDCVMCMaxAngCtrlOutTqLim_Nm]
  [VINP_ADASAngCtrlTqWeightGain_pct] -> LFCAOIControl/6(VINP_ADASAngCtrlTqWeightGain_pct)
  [VINP_VehicleType_enum] -> LFCAOIControl/10(VINP_VehicleType_enum)
  [VINP_ADASDrvInputTqBoostGain_pct] -> LFCAOIControl/9(VINP_ADASDrvInputTqBoostGain_pct)
  [VINP_ADASMaxAngCtrlOutTqLimit_Nm] -> LFCAOIControl/8(VINP_ADASMaxAngCtrlOutTqLimit_Nm)
  [VINP_ADASDesStrWhlAngCtrlCmd_Deg] -> LFCAOIControl/5(VINP_ADASDesStrWhlAngCtrlCmd_Deg)
  [VINP_APSAngleTarget_Deg] -> LFCAOIControl/4(VINP_APSAngleTarget_Deg)
  [VINP_ADASStrWhlAngCtrlStatus_flg] -> LFCAOIControl/3(VINP_ADASStrWhlAngCtrlStatus_flg)
  [VINP_APSRqEPASCtrl_flg] -> LFCAOIControl/2(VINP_APSRqEPASCtrl_flg)
  [VINP_ADASDrvInputTqBoostAct_flg] -> LFCAOIControl/7(VINP_ADASDrvInputTqBoostAct_flg)
  [VINP_APSVRqEPASCtrl_flg] -> LFCAOIControl/1(VINP_APSVRqEPASCtrl_flg)
  [VTQD_SWC1SetdownSta_flg] -> MSA function/28(VTQD_SWC1SetdownSta_flg)
  [VTQD_SWC1ResUpSta_flg] -> MSA function/27(VTQD_SWC1ResUpSta_flg)
  [VTQD_SWC1CANCELSta_flg] -> MSA function/26(VTQD_SWC1CANCELSta_flg)
  VTQD_SWC1SetdownSta_flg/1 -> [VTQD_SWC1SetdownSta_flg]
  VTQD_SWC1ResUpSta_flg/1 -> [VTQD_SWC1ResUpSta_flg]
  VTQD_SWC1CANCELSta_flg/1 -> [VTQD_SWC1CANCELSta_flg]
  [VTQD_EVDriveMode_enum] -> ACC_Function/47(VTQD_EVDriveMode_enum)
  VTQD_EVDriveMode_enum/1 -> [VTQD_EVDriveMode_enum]
  [VINP_SWCType_enum] -> MSA function/25(VINP_SWCType_enum)
  VINP_VehicleType_enum/1 -> [VINP_VehicleType_enum]
  VINP_SWCType_enum/1 -> [VINP_SWCType_enum]
  Equal2/1 -> Switch3/2
  [VINP_VehicleType_enum] -> Equal2/1
  Constant6/1 -> Equal2/2
  Equal1/1 -> Switch1/2
  Constant14/1 -> Equal1/2
  [VINP_VehicleType_enum] -> Equal1/1
  [VVMC_FDCVMCAngCtrlTqWtGn_pct] -> VVMC_FDCVMCAngCtrlTqWtGn_pct/1
  [VVMC_FDCVMCDrInpTqBstAct_flg] -> VVMC_FDCVMCDrInpTqBstAct_flg/1  "VVMC_FDCVMCDrInpTqBstAct_flg"
  [VVMC_FDCVMCMaxAngCtrlOutTqLim_Nm] -> VVMC_FDCVMCMaxAngCtrlOutTqLim_Nm/1  "VVMC_FDCVMCMaxAngCtrlOutTqLim_Nm"
  [VVMC_FDCVMCDrInpTqBstGn_pct] -> VVMC_FDCVMCDrInpTqBstGn_pct/1  "VVMC_FDCVMCDrInpTqBstGn_pct"
  VINP_APSVRqEPASCtrl_flg/1 -> [VINP_APSVRqEPASCtrl_flg]
  VINP_APSRqEPASCtrl_flg/1 -> [VINP_APSRqEPASCtrl_flg]
  VINP_APSAngleTarget_Deg/1 -> [VINP_APSAngleTarget_Deg]
  [VVMC_FDCVMCAPSAngleTarget_deg] -> VVMC_FDCVMCAPSAngleTarget_deg/1
  [VVMC_FDCVMCAPSRqEPSCtrl_flg] -> VVMC_FDCVMCAPSRqEPSCtrl_flg/1
  [VVMC_FDCVMCAPSVRqEPSCtrl_flg] -> VVMC_FDCVMCAPSVRqEPSCtrl_flg/1
  VINP_ADASDesStrWhlAngCtrlCmd_Deg/1 -> [VINP_ADASDesStrWhlAngCtrlCmd_Deg]
  VINP_ADASAngCtrlTqWeightGain_pct/1 -> [VINP_ADASAngCtrlTqWeightGain_pct]
  VINP_ADASDrvInputTqBoostGain_pct/1 -> [VINP_ADASDrvInputTqBoostGain_pct]
  VINP_ADASMaxAngCtrlOutTqLimit_Nm/1 -> [VINP_ADASMaxAngCtrlOutTqLimit_Nm]
  VINP_ADASStrWhlAngCtrlStatus_flg/1 -> [VINP_ADASStrWhlAngCtrlStatus_flg]
  VINP_ADASDrvInputTqBoostAct_flg/1 -> [VINP_ADASDrvInputTqBoostAct_flg]
  VINP_RrTMSpd_rpm/1 -> Switch3/1
  Switch3/1 -> [VINP_RrTMSpd_rpm]  "VINP_RrTMSpd_rpm"
  Switch1/1 -> [VINP_FrTMSpd_rpm]  "VINP_FrTMSpd_rpm"
  VINP_FrTMSpd_rpm/1 -> Switch1/1
  VINP_FrTMSpdNidec_rpm/1 -> Switch1/3
  [VINP_EPBSta_enum] -> SPD2ACC/31(VINP_EPBSta_enum)
  [VTQD_LowIdleAccPedal_flg] -> SPD2ACC/30(VTQD_LowIdleAccPedal_flg)
  [VTQD_GearActualPosn_enum] -> SPD2ACC/29(VTQD_GearActualPosn_enum)
  [VINP_BrkSwSta_flg] -> SPD2ACC/28(VINP_BrkSwSta_flg)
  SPD2ACC/13(VVMC_ACCShutOffHold_flg) -> [VVMC_ACCShutOffHold_flg]
  SPD2ACC/12(VVMC_ACCVehHoldReq_flg) -> [VVMC_ACCVehHoldReq_flg]
  SPD2ACC/11(VVMC_AccelTurnHold_flg) -> [VVMC_AccelTurnHold_flg]
  [VDSC_PreACC_flg] -> SpeedArbitration/20(VDSC_PreACC_flg)
  [VDSC_DISCSta_enum] -> SPD2ACC/25(VDSC_DISCSta_enum)
  [VDSC_PreACC_mps2] -> SPD2ACC/24(VDSC_PreACC_mps2)
  [VDSC_PreACC_flg] -> SPD2ACC/23(VDSC_PreACC_flg)
  [VDSC_AutoTurnMode_flg] -> SPD2ACC/26(VDSC_AutoTurnMode_flg)
  [VDSC_AccDecResp_flg] -> SPD2ACC/27(VDSC_AccDecResp_flg)
  [VDSC_TurningSpdMovingflat_kph] -> Switch2/1
  [VDSC_DISCSta_enum] -> Relational Operator8/1
  [VDSC_DISCTargetSpd_kph] -> Switch2/3  "VDSC_DISCTargetSpd_kph"
  Relational Operator8/1 -> AND9/2
  Constant15/1 -> Relational Operator8/2
  AND9/1 -> Switch2/2
  [VDSC_AutoTurnMode_flg] -> AND9/1
  VDSC_PreACC_flg/1 -> [VDSC_PreACC_flg]
  VDSC_PreACC_mps2/1 -> [VDSC_PreACC_mps2]
  VINP_APSVMCReqA_flg/1 -> [VINP_APSVMCReqA_flg]
  VINP_APSShiftPosnReq_enum/1 -> [VINP_APSShiftPosnReq_enum]
  [VVMC_VMCMSACtrlAvail_flg] -> MSA function/24(VVMC_VMCMSACtrlAvail_flg)
  [VVMC_VMCCCCtrlAvail_flg] -> CruiseControlFunction/25(VVMC_VMCCCCtrlAvail_flg)
  [VINP_ADASACCSta_enum] -> ACC_Function/46(VINP_ADASACCSta_enum)
  [VVMC_ACCShutOffHold_flg] -> ACC_Function/45(VVMC_ACCShutOffHold_flg)
  [VVMC_ACCShutOffHold_flg] -> VMC_FCM1/58(VVMC_ACCShutOffHold_flg)
  [VTQD_ExtDoorAllow_flg] -> CruiseControlFunction/24(VTQD_ExtDoorAllow_flg)
  [VVMC_AntiLimitSpd_kph] -> SpeedArbitration/19(VVMC_AntiLimitSpd_kph)
  MSA function/8(VVMC_AntiSpdLimSpdEn_flg) -> [VVMC_AntiSpdLimSpdEn_flg]
  MSA function/7(VVMC_AntiLimitSpd_kph) -> [VVMC_AntiLimitSpd_kph]
  [VVMC_APSActive_flg] -> MSA function/23(VVMC_APSActive_flg)
  [VINP_SmartEcoModeSW_flg] -> MSA function/22(VINP_SmartEcoModeSW_flg)
  VINP_SmartEcoModeSW_flg/1 -> [VINP_SmartEcoModeSW_flg]
  [VVMC_SetACCDisableAPS_flg] -> VVMC_SetACCDisableAPS_flg/1
  APS function/11(VVMC_SetACCDisableAPS_flg) -> [VVMC_SetACCDisableAPS_flg]
  VINP_IVISWCVibModeSta_enum/1 -> [VINP_IVISWCVibModeSta_enum]
  [VVMC_CalibratedAccZ_G] -> VVMC_CalibratedAccZ_G/1  "VVMC_CalibratedAccZ_G"
  [VVMC_CalibratedAccY_G] -> VVMC_CalibratedAccY_G/1  "VVMC_CalibratedAccY_G"
  [VVMC_CalibratedAccX_G] -> VVMC_CalibratedAccX_G/1  "VVMC_CalibratedAccX_G"
  [VVMC_CalibratedGyroZ_Dps] -> VVMC_CalibratedGyroZ_Dps/1  "VVMC_CalibratedGyroZ_Dps"
  [VVMC_CalibratedGyroX_Dps] -> VVMC_CalibratedGyroX_Dps/1  "VVMC_CalibratedGyroX_Dps"
  [VVMC_ExtraMSACtrlSta_enum] -> "VVMC_ExtraMSACtrlSta_enum "/1
  MSA function/6(VVMC_ExtraMSACtrlSta_enum) -> [VVMC_ExtraMSACtrlSta_enum]
  VINP_APSDecReqA_flg/1 -> [VINP_APSDecReqA_flg]
  VINP_APSDecReq_mps2/1 -> [VINP_APSDecReq_mps2]
  VINP_APSReq_enum/1 -> [VINP_APSReq_enum]
  VINP_CAASVMCReqA_flg/1 -> [VINP_CAASVMCReqA_flg]
  VINP_APSStaSystem_enum/1 -> [VINP_APSStaSystem_enum]
  [VVMC_CalibratedGyroY_Dps] -> VVMC_CalibratedGyroY_Dps/1  "VVMC_CalibratedGyroY_Dps"
  [VVMC_CAASActive_flg] -> VVMC_CAASActive_flg/1
  [VVMC_CAASCtrlAvail_flg] -> VVMC_CAASCtrlAvail_flg/1
  APS function/4(VVMC_CAASActive_flg) -> [VVMC_CAASActive_flg]
  APS function/5(VVMC_APSSpeedCMD_kph) -> [VVMC_APSSpeedCMD_kph]
  APS function/6(VVMC_APSShiftPosnReq_enum) -> [VVMC_APSShiftPosnReq_enum]
  APS function/7(VVMC_APSStaSys_enum) -> [VVMC_APSStaSys_enum]
  APS function/8(VVMC_APSDecReqA_flg) -> [VVMC_APSDecReqA_flg]
  APS function/9(VVMC_APSDecReq_mps2) -> [VVMC_APSDecReq_mps2]
  APS function/10(VVMC_APSReq_enum) -> [VVMC_APSReq_enum]
  APS function/3(VVMC_CAASCtrlAvail_flg) -> [VVMC_CAASCtrlAvail_flg]
  APS function/2(VVMC_APSActive_flg) -> [VVMC_APSActive_flg]
  APS function/1(VVMC_APSCtrlAvail_flg) -> [VVMC_APSCtrlAvail_flg]
  VTQD_VehActSpd_kph/1 -> [VTQD_VehActSpd_kph]
  [VTQD_RegenMode_enum] -> Slide Rate  Calculation/15(VTQD_RegenMode_enum)
  [VTQD_VehActSpd_kph] -> Slide Rate  Calculation/16(VTQD_VehActSpd_kph)
  [VVMC_EstSlope_Deg] -> Slide Rate  Calculation/17(VVMC_EstSlope_Deg)
  [VVMC_ACCOvrdMemTq_Nm] -> VVMC_ACCOvrdMemTq_Nm/1
  ACC_Function/10(VVMC_ACCOvrdMemTq_Nm) -> [VVMC_ACCOvrdMemTq_Nm]
  [VTQD_CreepBaseTqD_Nm] -> ACC_Function/44(VTQD_CreepBaseTqD_Nm)
  VTQD_CreepBaseTqD_Nm/1 -> [VTQD_CreepBaseTqD_Nm]
  [VINP_LongAccel_Gps] -> Switch8/3
  [VVMC_CalibratedAccX_G] -> Switch8/1
  Constant11/1 -> AND6/2
  [VVMC_IMUEnaCmd_flg] -> AND6/1
  AND6/1 -> Switch8/2
  [VINP_YawRate_degps] -> Switch7/3
  Constant10/1 -> AND5/2
  [VVMC_IMUEnaCmd_flg] -> AND5/1
  [VVMC_CalibratedGyroZ_Dps] -> Switch7/1
  AND5/1 -> Switch7/2
  [VINP_LatAccel_Gps] -> Switch6/3
  AND4/1 -> Switch6/2
  [VVMC_CalibratedAccY_G] -> Switch6/1
  [VVMC_IMUEnaCmd_flg] -> AND4/1
  Constant28/1 -> AND4/2
  [VDHP_ActAPSPosn_pct] -> ACC_Function/43(VDHP_ActAPSPosn_pct)
  IMU/7(VVMC_CalibratedAccZ_G) -> [VVMC_CalibratedAccZ_G]
  IMU/6(VVMC_CalibratedAccY_G) -> [VVMC_CalibratedAccY_G]
  IMU/5(VVMC_CalibratedAccX_G) -> [VVMC_CalibratedAccX_G]
  IMU/4(VVMC_CalibratedGyroZ_Dps) -> [VVMC_CalibratedGyroZ_Dps]
  IMU/3(VVMC_CalibratedGyroY_Dps) -> [VVMC_CalibratedGyroY_Dps]
  IMU/2(VVMC_CalibratedGyroX_Dps) -> [VVMC_CalibratedGyroX_Dps]
  [VINP_Distanceunit_flg] -> MSA function/21(VINP_Distanceunit_flg)
  [VINP_Distanceunit_flg] -> CruiseControlFunction/23(VINP_Distanceunit_flg)
  [VINP_SASAngle_Deg] -> ACC_Function/42(VINP_SASAngle_Deg)
  [VINP_DIDGetDynoMode_flg] -> Long Acceleration Calculation/7(VINP_DIDGetDynoMode_flg)
  [VINP_DIDGetDynoMode_flg] -> RDC Determination/11(VINP_DIDGetDynoMode_flg)
  VINP_DIDGetDynoMode_flg/1 -> [VINP_DIDGetDynoMode_flg]
  [VTQD_ExtDoorAllow_flg] -> ACC_Function/41(VTQD_ExtDoorAllow_flg)
  [VVMC_AntiSpdLimSpdEn_flg] -> SpeedArbitration/18(VVMC_AntiSpdLimSpdEn_flg)
  [VTQD_GearActualPosn_enum] -> MSA function/20(VTQD_GearActualPosn_enum)
  VINP_HoodSW_flg/1 -> [VINP_HoodSW_flg]
  [VINP_HoodSW_flg] -> MSA function/19(VINP_HoodSW_flg)
  [VVMC_ActStESCYaw_Dps] -> VVMC_ActStESCYaw_Dps/1
  [VVMC_RDCEnSlideRate_pct] -> VVMC_RDCEnSlideRate_pct/1
  RDC Determination/3(VVMC_ActStESCYaw_degps) -> [VVMC_ActStESCYaw_Dps]
  RDC Determination/2(VVMC_RDCEnSlideRate_pct) -> [VVMC_RDCEnSlideRate_pct]
  RDC Determination/1(VVMC_RWDRDCActive_enum) -> [VVMC_RWDRDCActive_enum]
  [VINP_RDCActive_enum] -> RDC Determination/10(VINP_RDCActive_enum)
  Switch7/1 -> RDC Determination/9(VINP_YawRate_degps)
  [VVMC_VehicleSpeed_kph] -> RDC Determination/8(VVMC_VehicleSpeed_kph)
  Switch6/1 -> RDC Determination/7(VINP_LatAccel_Gps)
  [VINP_SASAngle_Deg] -> RDC Determination/6(VINP_SASAngle_Deg)
  [VINP_ESCActive_flg] -> RDC Determination/5(VINP_ESCActive_flg)
  [VTQD_AfterAvailableTqDemRr_Nm] -> RDC Determination/4(VTQD_AfterAvailableTqDemRr_Nm)
  [VTQD_AfterAvailableTqDemFr_Nm] -> RDC Determination/3(VTQD_AfterAvailableTqDemFr_Nm)
  [VVMC_ActMaxSlideRate_pct] -> RDC Determination/2(VVMC_ActMaxSlideRate_pct)
  [task_time_s] -> RDC Determination/1(task_time_s)  "task_time_s"
  Slide Rate  Calculation/19(VVMC_AltWhlSlideRate_pct) -> [VVMC_AltWhlSlideRate_pct]
  Slide Rate  Calculation/18(VVMC_AltRWhlSlideRate_pct) -> [VVMC_AltRWhlSlideRate_pct]
  Slide Rate  Calculation/17(VVMC_AltLWhlSlideRate_pct) -> [VVMC_AltLWhlSlideRate_pct]
  Slide Rate  Calculation/16(VVMC_ActRRSlideRate_pct) -> [VVMC_ActRRSlideRate_pct]
  Slide Rate  Calculation/15(VVMC_ActLRSlideRate_pct) -> [VVMC_ActLRSlideRate_pct]
  Slide Rate  Calculation/14(VVMC_ActRFSlideRate_pct) -> [VVMC_ActRFSlideRate_pct]
  Slide Rate  Calculation/13(VVMC_ActLFSlideRate_pct) -> [VVMC_ActLFSlideRate_pct]
  Slide Rate  Calculation/12(VVMC_ActMaxSlideRate_pct) -> [VVMC_ActMaxSlideRate_pct]
  Slide Rate  Calculation/11(VVMC_4WhlSpdSlideRate_pct) -> [VVMC_4WhlSpdSlideRate_pct]
  Slide Rate  Calculation/10(VVMC_PredictVehSpd_kph) -> [VVMC_PredictVehSpd_kph]
  Slide Rate  Calculation/9(VVMC_RR4WhlSpdSlideRate_pct) -> [VVMC_RR4WhlSpdSlideRate_pct]
  Slide Rate  Calculation/8(VVMC_LR4WhlSpdSlideRate_pct) -> [VVMC_LR4WhlSpdSlideRate_pct]
  Slide Rate  Calculation/7(VVMC_RF4WhlSpdSlideRate_pct) -> [VVMC_RF4WhlSpdSlideRate_pct]
  Slide Rate  Calculation/6(VVMC_LF4WhlSpdSlideRate_pct) -> [VVMC_LF4WhlSpdSlideRate_pct]
  Slide Rate  Calculation/5(VVMC_RRWhlSpdSlideRate_pct) -> [VVMC_RRWhlSpdSlideRate_pct]
  Slide Rate  Calculation/4(VVMC_LRWhlSpdSlideRate_pct) -> [VVMC_LRWhlSpdSlideRate_pct]
  Slide Rate  Calculation/3(VVMC_RFWhlSpdSlideRate_pct) -> [VVMC_RFWhlSpdSlideRate_pct]
  Slide Rate  Calculation/2(VVMC_LFWhlSpdSlideRate_pct) -> [VVMC_LFWhlSpdSlideRate_pct]
  Slide Rate  Calculation/1(VVMC_RawWhlSpdSlideRate_pct) -> [VVMC_RawWhlSpdSlideRate_pct]
  [VVMC_LongAcc_Gps] -> Slide Rate  Calculation/9(VVMC_LongAcc_Gps)  "VVMC_LongAcc_Gps"
  Switch8/1 -> Slide Rate  Calculation/8(VINP_LongAccel_Gps)
  [VINP_LFRawWhlSpeed_kph] -> Slide Rate  Calculation/1(VINP_LFRawWhlSpeed_kph)
  [VINP_RFRawWhlSpeed_kph] -> Slide Rate  Calculation/2(VINP_RFRawWhlSpeed_kph)
  [VINP_LRRawWhlSpeed_kph] -> Slide Rate  Calculation/3(VINP_LRRawWhlSpeed_kph)
  [VINP_RRRawWhlSpeed_kph] -> Slide Rate  Calculation/4(VINP_RRRawWhlSpeed_kph)
  [VVMC_VehicleSpeed_kph] -> Slide Rate  Calculation/5(VVMC_VehicleSpeed_kph)
  [VINP_BrkPedalPos_pct] -> Slide Rate  Calculation/6(VINP_BrkPedalPos_pct)
  [VINP_BrkSwSta_flg] -> Slide Rate  Calculation/7(VINP_BrkSwSta_flg)
  [task_time_s] -> Slide Rate  Calculation/10(task_time_s)  "task_time_s"
  [VTQD_AfterAvailableTqDemFr_Nm] -> Slide Rate  Calculation/11(VTQD_AfterAvailableTqDemFr_Nm)
  [VTQD_AfterAvailableTqDemRr_Nm] -> Slide Rate  Calculation/12(VTQD_AfterAvailableTqDemRr_Nm)
  [VTQD_EquivAccPedalSWSta_flg] -> Slide Rate  Calculation/13(VTQD_EquivAccPedalSWSta_flg)
  [VTQD_GearActualPosn_enum] -> Slide Rate  Calculation/14(VTQD_GearActualPosn_enum)
  [VDSC_AutoTurnMode_flg] -> SpeedArbitration/17(VDSC_AutoTurnMode_flg)
  [VVMC_ADASACCSta_enum] -> ACC_Function/40(VVMC_ADASACCSta_enum)
  [VVMC_AccelTurnHold_flg] -> ACC_Function/39(VVMC_AccelTurnHold_flg)
  [VVMC_TotalAvailBrkRgnTq_Nm] -> MSA function/18(VVMC_TotalAvailBrkRgnTq_Nm)
  [VVMC_TotalAvailBrkRgnTq_Nm] -> CruiseControlFunction/22(VVMC_TotalAvailBrkRgnTq_Nm)
  [VVMC_TotalAvailBrkRgnTq_Nm] -> ACC_Function/38(VVMC_TotalAvailBrkRgnTq_Nm)
  Add/1 -> [VVMC_TotalAvailBrkRgnTq_Nm]
  [VTQD_FrEDUAvailBrkRgnTq_Nm] -> Add/1
  [VTQD_RrEDUAvailBrkRgnTq_Nm] -> Add/2
  Long Acceleration Calculation/2(VVMC_EstSlope_Deg) -> [VVMC_EstSlope_Deg]
  [VVMC_EstSlope_Deg] -> VVMC_EstSlope_Deg/1  "VVMC_EstSlope_Deg"
  BINP_IMU_outputs/1 -> [BINP_IMU_outputs]
  [VINP_MCPressure_bar] -> SPD2ACC/22(VINP_MCPressure_bar)
  [VVMC_ACCObjDist_m] -> SPD2ACC/21(VVMC_ACCObjDist_m)
  [VINP_LFWhlRotDir_enum] -> SPD2ACC/17(VINP_LFWhlRotDir_enum)
  [VINP_LRWhlRotDir_enum] -> SPD2ACC/18(VINP_LRWhlRotDir_enum)
  [VINP_RFWhlRotDir_enum] -> SPD2ACC/19(VINP_RFWhlRotDir_enum)
  [VINP_RRWhlRotDir_enum] -> SPD2ACC/20(VINP_RRWhlRotDir_enum)
  VINP_RRWhlRotDir_enum/1 -> [VINP_RRWhlRotDir_enum]
  VINP_LFWhlRotDir_enum/1 -> [VINP_LFWhlRotDir_enum]
  VINP_RFWhlRotDir_enum/1 -> [VINP_RFWhlRotDir_enum]
  VINP_LRWhlRotDir_enum/1 -> [VINP_LRWhlRotDir_enum]
  [VINP_GRADE_Deg] -> SPD2ACC/16(VINP_GRADE_Deg)
  [task_time_s] -> IMU/13(task_time_s)  "task_time_s"
  [VDSC_AccDecResp_flg] -> SpeedArbitration/16(VDSC_AccDecResp_flg)
  Constant109/1 -> Switch5/1
  [VDSC_AutoTurnMode_flg] -> Switch5/2
  Switch4/1 -> Cast To Single31/1
  Constant7/1 -> Switch4/1
  [VDSC_AutoTurnMode_flg] -> Switch4/2
  VDSC_AccDecResp_flg/1 -> [VDSC_AccDecResp_flg]
  VDSC_AutoTurnMode_flg/1 -> [VDSC_AutoTurnMode_flg]
  VDSC_TurningSpdMovingflat_kph/1 -> [VDSC_TurningSpdMovingflat_kph]
  [VVMC_MSAWhlTqActive_flg] -> VVMC_MSAWhlTqActive_flg/1
  MSA function/5(VVMC_MSAWhlTqActive_flg) -> [VVMC_MSAWhlTqActive_flg]
  [VVMC_IMUEnaCmd_flg] -> VVMC_IMUEnaCmd_flg/1
  [VVMC_RWDRDCActive_enum] -> VVMC_RWDRDCActive_enum/1
  VINP_RDCActive_enum/1 -> [VINP_RDCActive_enum]
  VINP_YawRate_degps/1 -> [VINP_YawRate_degps]
  VINP_ESCActive_flg/1 -> [VINP_ESCActive_flg]
  Bus Selector10/5 -> IMU/5(VINP_MemOffsetAccY_raw16)  "<VINP_MemOffsetAccY_raw16>"
  Bus Selector10/10 -> IMU/10(VINP_SensingAccX_raw16)  "<VINP_SensingAccX_raw16>"
  Bus Selector10/6 -> IMU/6(VINP_MemOffsetAccZ_raw16)  "<VINP_MemOffsetAccZ_raw16>"
  Bus Selector10/4 -> IMU/4(VINP_MemOffsetAccX_raw16)  "<VINP_MemOffsetAccX_raw16>"
  Bus Selector10/7 -> IMU/7(VINP_SensingGyroX_raw16)  "<VINP_SensingGyroX_raw16>"
  [BINP_IMU_outputs] -> Bus Selector10/1
  Bus Selector10/3 -> IMU/3(VINP_MemOffsetGyroZ_raw16)  "<VINP_MemOffsetGyroZ_raw16>"
  Bus Selector10/8 -> IMU/8(VINP_SensingGyroY_raw16)  "<VINP_SensingGyroY_raw16>"
  Bus Selector10/2 -> IMU/2(VINP_MemOffsetGyroY_raw16)  "<VINP_MemOffsetGyroY_raw16>"
  Bus Selector10/1 -> IMU/1(VINP_MemOffsetGyroX_raw16)  "<VINP_MemOffsetGyroX_raw16>"
  Bus Selector10/12 -> IMU/12(VINP_SensingAccZ_raw16)  "<VINP_SensingAccZ_raw16>"
  Bus Selector10/9 -> IMU/9(VINP_SensingGyroZ_raw16)  "<VINP_SensingGyroZ_raw16>"
  IMU/1(VVMC_IMUEnaCmd_flg) -> [VVMC_IMUEnaCmd_flg]
  Bus Selector10/11 -> IMU/11(VINP_SensingAccY_raw16)  "<VINP_SensingAccY_raw16>"
  VTQD_ExtDoorAllow_flg/1 -> [VTQD_ExtDoorAllow_flg]
  Switch5/1 -> Cast To Single34/1
  [VINP_Distanceunit_flg] -> FeatureSetSpeed/5(VINP_Distanceunit_flg)  "VINP_Distanceunit_flg"
  Unit Delay8/1 -> MSA function/17(VTQR_RrTMTqReq_Nm)
  Unit Delay7/1 -> MSA function/16(VTQR_FrTMTqReq_Nm)
  Unit Delay6/1 -> CruiseControlFunction/18(VTQR_RrTMTqReq_Nm)
  Unit Delay5/1 -> CruiseControlFunction/17(VTQR_FrTMTqReq_Nm)
  [VTQR_RrTMTqReq_Nm] -> Unit Delay8/1
  [VTQR_FrTMTqReq_Nm] -> Unit Delay7/1
  [VVMC_ActACCRequiredAccel_mps2] -> MSA function/15(VVMC_ActACCRequiredAccel_mps2)
  VMC_FCM1/11(VVMC_ADASACCSta_enum) -> [VVMC_ADASACCSta_enum]  "VVMC_ADASACCSta_enum"
  VMC_FCM1/9(VVMC_ACCVehHoldReqRaw_flg) -> [VVMC_ACCVehHoldReqRaw_flg]  "VVMC_ACCVehHoldReqRaw_flg"
  [VPMM_DrivetrainSelect_enum] -> ACC_Function/37(VPMM_DrivetrainSelect_enum)
  <VPMM_DrivetrainSelect_enum>/1 -> [VPMM_DrivetrainSelect_enum]
  VINP_SASAngle_Deg/1 -> [VINP_SASAngle_Deg]
  [VVMC_ActACCRequiredAccel_mps2] -> CruiseControlFunction/20(VVMC_ActACCRequiredAccel_mps2)
  [task_time_s] -> CruiseControlFunction/21(task_time_s)
  [VTQD_RegenMode_enum] -> CruiseControlFunction/19(VTQD_RegenMode_enum)
  [VTQR_RrTMTqReq_Nm] -> Unit Delay6/1
  [VTQR_FrTMTqReq_Nm] -> Unit Delay5/1
  [VVMC_SafetyCtrl_flg] -> CruiseControlFunction/16(VVMC_SafetyCtrl_flg)
  [VVMC_ACCLowSpdTqCtrl_flg] -> SPD2ACC/15(VVMC_ACCLowSpdTqCtrl_flg)
  ACC_Function/9(VVMC_ACCLowSpdTqCtrl_flg) -> [VVMC_ACCLowSpdTqCtrl_flg]
  [VTQD_FrEDUAvailBrkRgnTq_Nm] -> ACC_Function/36(VTQD_FrEDUAvailBrkRgnTq_Nm)
  [VTQD_RrEDUAvailBrkRgnTq_Nm] -> ACC_Function/35(VTQD_RrEDUAvailBrkRgnTq_Nm)  "VTQD_RrEDUAvailBrkRgnTq_Nm"
  VTQD_FrEDUAvailBrkRgnTq_Nm/1 -> [VTQD_FrEDUAvailBrkRgnTq_Nm]
  VTQR_FrTMTqReq_Nm/1 -> [VTQR_FrTMTqReq_Nm]
  [VTQR_FrTMTqReq_Nm] -> ACC_Function/34(VTQR_FrTMTqReq_Nm)
  SPD2ACC/10(VVMC_VehHoldDecCtrlHEnd_flg) -> Terminator2/1
  [VVMC_EstSlope_Deg] -> SPD2ACC/14(VVMC_EstSlope_Deg)
  [VVMC_ACCVehHoldReqRaw_flg] -> SPD2ACC/13(VVMC_ACCVehHoldReqRaw_flg)
  [VVMC_CCMSASpdWar_flg] -> VVMC_CCMSASpdWar_flg/1
  [VVMC_AltRWhlSlideRate_pct] -> VVMC_AltRWhlSlideRate_pct/1
  [VVMC_AltWhlSlideRate_pct] -> VVMC_AltWhlSlideRate_pct/1
  [VVMC_ActRRSlideRate_pct] -> VVMC_ActRRSlideRate_pct/1  "VVMC_ActRRSlideRate_pct"
  [VVMC_AltLWhlSlideRate_pct] -> VVMC_AltLWhlSlideRate_pct/1
  [VVMC_RR4WhlSpdSlideRate_pct] -> VVMC_RR4WhlSpdSlideRate_pct/1
  [VVMC_ActLRSlideRate_pct] -> VVMC_ActLRSlideRate_pct/1  "VVMC_ActLRSlideRate_pct"
  [VVMC_ActLFSlideRate_pct] -> VVMC_ActLFSlideRate_pct/1  "VVMC_ActLFSlideRate_pct"
  [VVMC_RF4WhlSpdSlideRate_pct] -> VVMC_RF4WhlSpdSlideRate_pct/1
  [VVMC_PredictVehSpd_kph] -> VVMC_PredictVehSpd_kph/1
  [VVMC_ActMaxSlideRate_pct] -> VVMC_ActMaxSlideRate_pct/1  "VVMC_ActMaxSlideRate_pct"
  [VVMC_LF4WhlSpdSlideRate_pct] -> VVMC_LF4WhlSpdSlideRate_pct/1
  [VVMC_LR4WhlSpdSlideRate_pct] -> VVMC_LR4WhlSpdSlideRate_pct/1
  [VVMC_ActRFSlideRate_pct] -> VVMC_ActRFSlideRate_pct/1  "VVMC_ActRFSlideRate_pct"
  [VVMC_4WhlSpdSlideRate_pct] -> VVMC_4WhlSpdSlideRate_pct/1
  [VVMC_LFWhlSpdSlideRate_pct] -> VVMC_LFWhlSpdSlideRate_pct/1
  [VVMC_RawWhlSpdSlideRate_pct] -> VVMC_RawWhlSpdSlideRate_pct/1
  [VVMC_RRWhlSpdSlideRate_pct] -> VVMC_RRWhlSpdSlideRate_pct/1
  [VVMC_LRWhlSpdSlideRate_pct] -> VVMC_LRWhlSpdSlideRate_pct/1
  [VVMC_RFWhlSpdSlideRate_pct] -> VVMC_RFWhlSpdSlideRate_pct/1
  [VVMC_LongAcc_Gps] -> VVMC_LongAcc_Gps/1  "VVMC_LongAcc_Gps"
  [VVMC_APSDecReqA_flg] -> VVMC_APSDecReqA_flg/1
  [VVMC_APSStaSys_enum] -> VVMC_APSStaSys_enum/1
  [VVMC_APSReq_enum] -> VVMC_APSReq_enum/1
  [VVMC_APSDecReq_mps2] -> VVMC_APSDecReq_mps2/1
  [VVMC_MSAActive_flg] -> VVMC_MSAActive_flg/1
  [VVMC_MSACtrlSta_enum] -> VVMC_MSACtrlSta_enum/1
  [VVMC_MSAWhlTqReq_Nm] -> VVMC_MSAWhlTqReq_Nm/1
  [VVMC_CCPedalOvrd_flg] -> VVMC_CCPedalOvrd_flg/1  "VVMC_CCPedalOvrd_flg"
  [VVMC_CCCtrlSta_enum] -> VVMC_CCCtrlSta_enum/1
  [VVMC_CruzWhlTqReq_Nm] -> VVMC_CruzWhlTqReq_Nm/1  "VVMC_CruzWhlTqReq_Nm"
  [VVMC_CruzActive_flg] -> VVMC_CruzActive_flg/1
  [VVMC_TimeGapCalcu_s] -> VVMC_TimeGapCalcu_s/1
  [VVMC_RearTqRatio_rat] -> VVMC_RearTqRatio_rat/1
  [VVMC_AccPedalOvrdDISC_flg] -> VVMC_AccPedalOvrdDISC_flg/1
  [VVMC_ADASWhlTqReq_Nm] -> VVMC_ADASWhlTqReq_Nm/1
  [VVMC_ACCPedalOvrd_flg] -> VVMC_ACCPedalOvrd_flg/1
  [VVMC_ADASNegReq_flg] -> VVMC_ADASNegReq_flg/1
  [VVMC_FCMLDWFault_flg] -> VVMC_FCMLDWFault_flg/1
  [VVMC_FCMLDWRequest_enum] -> VVMC_FCMLDWRequest_enum/1
  [VVMC_ADASAEBReq_enum] -> VVMC_ADASAEBReq_enum/1
  [VVMC_ADASLanecurveL_raw32] -> VVMC_ADASLanecurveL_raw32/1
  [VVMC_ADASLFCWarnSound_enum] -> VVMC_ADASLFCWarnSound_enum/1
  [VVMC_ADASLanetypeL_enum] -> VVMC_ADASLanetypeL_enum/1
  [VVMC_ADASLanecurveR_raw32] -> VVMC_ADASLanecurveR_raw32/1
  [VVMC_ADASLanetypeR_enum] -> VVMC_ADASLanetypeR_enum/1
  [VVMC_FCMACCmode_enum] -> VVMC_FCMACCmode_enum/1
  [VVMC_LVDAWarning_flg] -> VVMC_LVDAWarning_flg/1
  [VVMC_LVDAACCStatusInformation_flg] -> VVMC_LVDAACCStatusInformation_flg/1
  [VVMC_LVDAFailinfo_flg] -> VVMC_LVDAFailinfo_flg/1
  [VVMC_LVDAMuteSta_enum] -> VVMC_LVDAMuteSta_enum/1
  [VVMC_LVDADisabled_flg] -> VVMC_LVDADisabled_flg/1
  [VVMC_ADASLFCHandsOffWarning_enum] -> VVMC_ADASLFCHandsOffWarning_enum/1
  [VVMC_ADASLaneModeL_enum] -> VVMC_ADASLaneModeL_enum/1
  [VVMC_ADASLaneModeR_enum] -> VVMC_ADASLaneModeR_enum/1
  [VVMC_ADASSLIFSta_enum] -> VVMC_ADASSLIFSta_enum/1
  [VVMC_ADASFCWMute_flg] -> VVMC_ADASFCWMute_flg/1
  [VVMC_ADASLDWMute_flg] -> VVMC_ADASLDWMute_flg/1
  [VVMC_ADASISASta_enum] -> VVMC_ADASISASta_enum/1
  [VVMC_ADASLFCSta_enum] -> VVMC_ADASLFCSta_enum/1
  [VVMC_TargetType_enum] -> VVMC_TargetType_enum/1
  [VVMC_LKAHODDisplayWarning_flg] -> VVMC_LKAHODDisplayWarning_flg/1
  [VVMC_ADASSLIFSpdLim_enum] -> VVMC_ADASSLIFSpdLim_enum/1
  [VVMC_ADASWarningMsg_enum] -> VVMC_ADASWarningMsg_enum/1
  [VVMC_ADASCAMSpdLim_enum] -> VVMC_ADASCAMSpdLim_enum/1
  [VVMC_LKAHODSoundWarning_flg] -> VVMC_LKAHODSoundWarning_flg/1
  [VVMC_ACCObjDstLvl_enum] -> VVMC_ACCObjDstLvl_enum/1
  [VVMC_ForceLowBeam_enum] -> VVMC_ForceLowBeam_enum/1
  [VVMC_ACCTakeoverReq_flg] -> VVMC_ACCTakeoverReq_flg/1
  [VVMC_ADASLDWSta_enum] -> VVMC_ADASLDWSta_enum/1
  [VVMC_ADASFCWSta_enum] -> VVMC_ADASFCWSta_enum/1
  [VVMC_ADASFltWrnReq_flg] -> VVMC_ADASFltWrnReq_flg/1
  [VVMC_RightTurnLightReq_flg] -> VVMC_RightTurnLightReq_flg/1
  [VVMC_HazardWarningReq_flg] -> VVMC_HazardWarningReq_flg/1
  [VVMC_LeftTurnLightReq_flg] -> VVMC_LeftTurnLightReq_flg/1
  [VVMC_ADASForceIdle_flg] -> VVMC_ADASForceIdle_flg/1
  [VVMC_ADASShftPosnReq_enum] -> VVMC_ADASShftPosnReq_enum/1
  [VVMC_ADASShftPosnReqA_flg] -> VVMC_ADASShftPosnReqA_flg/1
  [VVMC_ADASVehSpdLim_raw32] -> VVMC_ADASVehSpdLim_raw32/1
  [VVMC_ACCComfortBandUpper_mps2] -> VVMC_ACCComfortBandUpper_mps2/1
  [VVMC_ACCJerkUpperLimit_mps3] -> VVMC_ACCJerkUpperLimit_mps3/1
  [VVMC_ACCComfortBandLower_mps2] -> VVMC_ACCComfortBandLower_mps2/1
  [VVMC_ACCJerkLowerLimit_mps3] -> VVMC_ACCJerkLowerLimit_mps3/1
  [VVMC_TimeGapLevel_enum] -> VVMC_TimeGapLevel_enum/1
  [VVMC_ACCObjDist_m] -> VVMC_ACCObjDist_m/1
  [VVMC_ACCObjRelSpd_mps] -> VVMC_ACCObjRelSpd_mps/1
  [VVMC_ADASACCSta_enum] -> VVMC_ADASACCSta_enum/1  "VVMC_ADASACCSta_enum"
  [VVMC_ADASDBSReq_enum] -> VVMC_ADASDBSReq_enum/1
  [VVMC_ACCVehHoldReq_flg] -> VVMC_ACCVehHoldReq_flg/1  "VVMC_ACCVehHoldReq_flg"
  [VVMC_ADASFaultSta_flg] -> VVMC_ADASFaultSta_flg/1
  [VVMC_ADASAEBSta_enum] -> VVMC_ADASAEBSta_enum/1
  [VVMC_LKATOIFault_flg] -> VVMC_LKATOIFault_flg/1
  [VVMC_LKAStrToqReq_Nm] -> VVMC_LKAStrToqReq_Nm/1
  [VVMC_LKATOIAct_enum] -> VVMC_LKATOIAct_enum/1
  [VVMC_ADASLKASta_enum] -> VVMC_ADASLKASta_enum/1
  [VVMC_LateralCtrl_flg] -> VVMC_LateralCtrl_flg/1
  [VVMC_FeatArbitrFinal_enum] -> VVMC_FeatArbitrFinal_enum/1
  [VVMC_ActACCRequiredAccel_mps2] -> VVMC_ActACCRequiredAccel_mps2/1
  [VVMC_ACCRequiredAccel_mps2] -> VVMC_ACCRequiredAccel_mps2/1
  [VVMC_DISCReqAcc_mps2] -> VVMC_DISCReqAcc_mps2/1  "VVMC_DISCReqAcc_mps2"
  [VVMC_ISODecLimit_mps2] -> VVMC_ISODecLimit_mps2/1
  [VVMC_AccCalcuPID_mps2] -> VVMC_AccCalcuPID_mps2/1
  [VVMC_ISOAccLimit_mps2] -> VVMC_ISOAccLimit_mps2/1
  [VVMC_SPD2ACCAct_flg] -> VVMC_SPD2ACCAct_flg/1
  [VVMC_ISOJerkLimit_mps3] -> VVMC_ISOJerkLimit_mps3/1
  [VVMC_SafetyCtrl_flg] -> VVMC_SafetyCtrl_flg/1
  [VVMC_SingleWhlSlipRatioCtrl_flg] -> VVMC_SingleWhlSlipRatioCtrl_flg/1
  [VVMC_FrontRearSlipRatioCtrl_flg] -> VVMC_FrontRearSlipRatioCtrl_flg/1
  [VVMC_RearWhlSlipRatioCtrl_flg] -> VVMC_RearWhlSlipRatioCtrl_flg/1
  [VVMC_LatAccCtrl_flg] -> VVMC_LatAccCtrl_flg/1
  [VVMC_LRWhlSpeedRollAve_kph] -> VVMC_LRWhlSpeedRollAve_kph/1  "VVMC_LRWhlSpeedRollAve_kph"
  [VVMC_RRWhlSpeedRollAve_kph] -> VVMC_RRWhlSpeedRollAve_kph/1  "VVMC_RRWhlSpeedRollAve_kph"
  [VVMC_RFWhlSpeedRollAve_kph] -> VVMC_RFWhlSpeedRollAve_kph/1  "VVMC_RFWhlSpeedRollAve_kph"
  [VVMC_LFWhlSpeedRollAve_kph] -> VVMC_LFWhlSpeedRollAve_kph/1  "VVMC_LFWhlSpeedRollAve_kph"
  [VVMC_FeatReqSpd_kph] -> VVMC_FeatReqSpd_kph/1
  [VVMC_FeatArbitrSta_enum] -> VVMC_FeatArbitrSta_enum/1  "VVMC_FeatArbitrSta_enum"
  [VVMC_LimitPCT_pct] -> VVMC_LimitPCT_pct/1
  [VVMC_JerkPCT_pct] -> VVMC_JerkPCT_pct/1
  [VVMC_VMCAEBCtrlAvail_flg] -> VVMC_VMCAEBCtrlAvail_flg/1
  [VVMC_VMCMSACtrlAvail_flg] -> VVMC_VMCMSACtrlAvail_flg/1
  [VVMC_VMCCCCtrlAvail_flg] -> VVMC_VMCCCCtrlAvail_flg/1
  [VVMC_VMCACCCtrlAvail_flg] -> VVMC_VMCACCCtrlAvail_flg/1
  [VVMC_MeterIndSpeedForCalcu_kph] -> VVMC_MeterIndSpeedForCalcu_kph/1
  [VVMC_MeterIndSpeed_raw32] -> VVMC_MeterIndSpeed_raw32/1
  [VVMC_VehicleSpeed_kph] -> VVMC_VehicleSpeed_kph/1
  [VVMC_VehicleSpeed_mph] -> VVMC_VehicleSpeed_mph/1
  [VVMC_MSAActive_flg] -> ACC_Function/33(VVMC_MSAActive_flg)
  [VVMC_MSAWhlTqReq_Nm] -> ACC_Function/32(VVMC_MSAWhlTqReq_Nm)
  [VVMC_CruzActive_flg] -> ACC_Function/31(VVMC_CruzActive_flg)
  [VVMC_CruzWhlTqReq_Nm] -> ACC_Function/30(VVMC_CruzWhlTqReq_Nm)
  [VVMC_FrRrSlipSpd_kph] -> ACC_Function/29(VVMC_FrRrSlipSpd_kph)
  [VINP_LongAccel_Gps] -> ACC_Function/28(VINP_LongAccel_Gps)  "VINP_LongAccel_Gps"
  ACC_Function/8(VVMC_RearTqRatio_rat) -> [VVMC_RearTqRatio_rat]
  [VVMC_SafetyCtrl_flg] -> ACC_Function/27(VVMC_SafetyCtrl_flg)
  [VINP_TargetType_enum] -> ACC_Function/26(VINP_TargetType_enum)
  [VVMC_LongAccelCalcuByVehSpdRaw_gps] -> Long Acceleration Calculation/6(VVMC_LongAccelCalcuByVehSpdRaw_gps)
  VTQD_AfterAvailableTqDemFr_Nm/1 -> [VTQD_AfterAvailableTqDemFr_Nm]
  VTQD_AfterAvailableTqDemRr_Nm/1 -> [VTQD_AfterAvailableTqDemRr_Nm]
  VTQD_EquivAccPedalSWSta_flg/1 -> [VTQD_EquivAccPedalSWSta_flg]
  VTQD_APSStaSys_enum/1 -> [VTQD_APSStaSys_enum]
  VTQD_APSDecReqA_flg/1 -> [VTQD_APSDecReqA_flg]
  VTQD_APSDecReq_mps2/1 -> [VTQD_APSDecReq_mps2]
  VTQD_APSReq_enum/1 -> [VTQD_APSReq_enum]
  [task_time_s] -> MSA function/14(task_time_s)  "task_time_s"
  [VDHP_ActAPSPosn_pct] -> MSA function/13(VDHP_ActAPSPosn_pct)  "VDHP_ActAPSPosn_pct"
  [VTQD_LowIdleAccPedal_flg] -> MSA function/12(VTQD_LowIdleAccPedal_flg)  "VTQD_LowIdleAccPedal_flg"
  VDHP_ActAPSPosn_pct/1 -> [VDHP_ActAPSPosn_pct]
  [VVMC_MeterIndSpeedForCalcu_kph] -> MSA function/11(VVMC_MeterIndSpeedForCalcu_kph)
  [VVMC_EstSlopeCal_Deg] -> Long Acceleration Calculation/5(VVMC_EstSlopeCal_Deg)
  [VVMC_EstSlope_Deg] -> ACC_Function/25(VVMC_EstSlope_Deg)
  SPD2ACC/9(VVMC_ActACCRequiredAccel_mps2) -> [VVMC_ActACCRequiredAccel_mps2]
  VTQD_RrEDUAvailBrkRgnTq_Nm/1 -> [VTQD_RrEDUAvailBrkRgnTq_Nm]
  Unit Delay1/1 -> SPD2ACC/12(VVMC_LastADASWhlTqReq_Nm)  "VVMC_LastADASWhlTqReq_Nm"
  [VVMC_ADASWhlTqReq_Nm] -> Unit Delay1/1
  VINP_BrkPedalPos_pct/1 -> [VINP_BrkPedalPos_pct]
  VMC_FCM1/59(VVMC_FCMLDWFault_flg) -> [VVMC_FCMLDWFault_flg]
  VMC_FCM1/58(VVMC_FCMLDWRequest_enum) -> [VVMC_FCMLDWRequest_enum]
  [VVMC_ACCVehHoldReqRaw_flg] -> ACC_Function/24(VVMC_ACCVehHoldReqRaw_flg)
  Function-Call Split/1 -> [Trigger_10ms_1]
  Scheduler/1(Trigger_10ms_1()) -> Function-Call Split/1
  Function-Call Split/2 -> [Trigger_10ms_2]
  VMC_FCM1/57(VVMC_ADASAEBSta_enum) -> [VVMC_ADASAEBSta_enum]  "VVMC_ADASAEBSta_enum"
  [VINP_ADASAEBSta_enum] -> VMC_FCM1/57(VINP_ADASAEBSta_enum)  "VINP_ADASAEBSta_enum"
  VMC_FCM1/56(VVMC_ADASLanecurveR_raw32) -> [VVMC_ADASLanecurveR_raw32]  "VVMC_ADASLanecurveR_raw32"
  VMC_FCM1/55(VVMC_ADASLanecurveL_raw32) -> [VVMC_ADASLanecurveL_raw32]  "VVMC_ADASLanecurveL_raw32"
  VMC_FCM1/54(VVMC_ADASLanetypeL_enum) -> [VVMC_ADASLanetypeL_enum]  "VVMC_ADASLanetypeL_enum"
  VMC_FCM1/53(VVMC_ADASLanetypeR_enum) -> [VVMC_ADASLanetypeR_enum]  "VVMC_ADASLanetypeR_enum"
  VMC_FCM1/52(VVMC_FCMACCmode_enum) -> [VVMC_FCMACCmode_enum]  "VVMC_FCMACCmode_enum"
  VMC_FCM1/51(VVMC_ADASLFCWarnSound_enum) -> [VVMC_ADASLFCWarnSound_enum]  "VVMC_ADASLFCWarnSound_enum"
  VMC_FCM1/50(VVMC_LVDAACCStatusInformation_flg) -> [VVMC_LVDAACCStatusInformation_flg]  "VVMC_LVDAACCStatusInformation_flg"
  VMC_FCM1/49(VVMC_LVDAWarning_flg) -> [VVMC_LVDAWarning_flg]  "VVMC_LVDAWarning_flg"
  VMC_FCM1/48(VVMC_LVDAFailinfo_flg) -> [VVMC_LVDAFailinfo_flg]  "VVMC_LVDAFailinfo_flg"
  VMC_FCM1/47(VVMC_LVDAMuteSta_enum) -> [VVMC_LVDAMuteSta_enum]  "VVMC_LVDAMuteSta_enum"
  VMC_FCM1/46(VVMC_LVDADisabled_flg) -> [VVMC_LVDADisabled_flg]  "VVMC_LVDADisabled_flg"
  VMC_FCM1/45(VVMC_ADASLFCHandsOffWarning_enum) -> [VVMC_ADASLFCHandsOffWarning_enum]  "VVMC_ADASLFCHandsOffWarning_enum"
  VMC_FCM1/44(VVMC_ADASFCWMute_flg) -> [VVMC_ADASFCWMute_flg]  "VVMC_ADASFCWMute_flg"
  VMC_FCM1/43(VVMC_ADASLDWMute_flg) -> [VVMC_ADASLDWMute_flg]  "VVMC_ADASLDWMute_flg"
  VMC_FCM1/42(VVMC_ADASISASta_enum) -> [VVMC_ADASISASta_enum]  "VVMC_ADASISASta_enum"
  VMC_FCM1/41(VVMC_ADASSLIFSta_enum) -> [VVMC_ADASSLIFSta_enum]  "VVMC_ADASSLIFSta_enum"
  VMC_FCM1/40(VVMC_ADASLaneModeR_enum) -> [VVMC_ADASLaneModeR_enum]  "VVMC_ADASLaneModeR_enum"
  VMC_FCM1/39(VVMC_ADASLaneModeL_enum) -> [VVMC_ADASLaneModeL_enum]  "VVMC_ADASLaneModeL_enum"
  VMC_FCM1/38(VVMC_ADASLFCSta_enum) -> [VVMC_ADASLFCSta_enum]  "VVMC_ADASLFCSta_enum"
  VMC_FCM1/37(VVMC_LKAHODSoundWarning_flg) -> [VVMC_LKAHODSoundWarning_flg]  "VVMC_LKAHODSoundWarning_flg"
  VMC_FCM1/36(VVMC_LKAHODDisplayWarning_flg) -> [VVMC_LKAHODDisplayWarning_flg]  "VVMC_LKAHODDisplayWarning_flg"
  VMC_FCM1/35(VVMC_ADASSLIFSpdLim_enum) -> [VVMC_ADASSLIFSpdLim_enum]  "VVMC_ADASSLIFSpdLim_enum"
  VMC_FCM1/34(VVMC_TargetType_enum) -> [VVMC_TargetType_enum]  "VVMC_TargetType_enum"
  VMC_FCM1/33(VVMC_ADASCAMSpdLim_enum) -> [VVMC_ADASCAMSpdLim_enum]  "VVMC_ADASCAMSpdLim_enum"
  VMC_FCM1/32(VVMC_ADASWarningMsg_enum) -> [VVMC_ADASWarningMsg_enum]  "VVMC_ADASWarningMsg_enum"
  VMC_FCM1/31(VVMC_ACCTakeoverReq_flg) -> [VVMC_ACCTakeoverReq_flg]  "VVMC_ACCTakeoverReq_flg"
  VMC_FCM1/30(VVMC_ForceLowBeam_enum) -> [VVMC_ForceLowBeam_enum]  "VVMC_ForceLowBeam_enum"
  VMC_FCM1/29(VVMC_ACCObjDstLvl_enum) -> [VVMC_ACCObjDstLvl_enum]  "VVMC_ACCObjDstLvl_enum"
  VMC_FCM1/28(VVMC_ADASFltWrnReq_flg) -> [VVMC_ADASFltWrnReq_flg]  "VVMC_ADASFltWrnReq_flg"
  VMC_FCM1/27(VVMC_ADASLDWSta_enum) -> [VVMC_ADASLDWSta_enum]  "VVMC_ADASLDWSta_enum"
  VMC_FCM1/26(VVMC_ADASFCWSta_enum) -> [VVMC_ADASFCWSta_enum]  "VVMC_ADASFCWSta_enum"
  VMC_FCM1/25(VVMC_LeftTurnLightReq_flg) -> [VVMC_LeftTurnLightReq_flg]  "VVMC_LeftTurnLightReq_flg"
  VMC_FCM1/24(VVMC_RightTurnLightReq_flg) -> [VVMC_RightTurnLightReq_flg]  "VVMC_RightTurnLightReq_flg"
  VMC_FCM1/23(VVMC_HazardWarningReq_flg) -> [VVMC_HazardWarningReq_flg]  "VVMC_HazardWarningReq_flg"
  VMC_FCM1/22(VVMC_ADASForceIdle_flg) -> [VVMC_ADASForceIdle_flg]  "VVMC_ADASForceIdle_flg"
  VMC_FCM1/21(VVMC_ADASShftPosnReq_enum) -> [VVMC_ADASShftPosnReq_enum]  "VVMC_ADASShftPosnReq_enum"
  VMC_FCM1/20(VVMC_ADASShftPosnReqA_flg) -> [VVMC_ADASShftPosnReqA_flg]  "VVMC_ADASShftPosnReqA_flg"
  VMC_FCM1/19(VVMC_ADASVehSpdLim_raw32) -> [VVMC_ADASVehSpdLim_raw32]  "VVMC_ADASVehSpdLim_raw32"
  VMC_FCM1/18(VVMC_ACCComfortBandLower_mps2) -> [VVMC_ACCComfortBandLower_mps2]  "VVMC_ACCComfortBandLower_mps2"
  VMC_FCM1/17(VVMC_ACCJerkLowerLimit_mps3) -> [VVMC_ACCJerkLowerLimit_mps3]  "VVMC_ACCJerkLowerLimit_mps3"
  VMC_FCM1/16(VVMC_ACCComfortBandUpper_mps2) -> [VVMC_ACCComfortBandUpper_mps2]  "VVMC_ACCComfortBandUpper_mps2"
  VMC_FCM1/15(VVMC_ACCJerkUpperLimit_mps3) -> [VVMC_ACCJerkUpperLimit_mps3]  "VVMC_ACCJerkUpperLimit_mps3"
  VMC_FCM1/14(VVMC_TimeGapLevel_enum) -> [VVMC_TimeGapLevel_enum]  "VVMC_TimeGapLevel_enum"
  VMC_FCM1/13(VVMC_ACCObjRelSpd_mps) -> [VVMC_ACCObjRelSpd_mps]  "VVMC_ACCObjRelSpd_mps"
  VMC_FCM1/12(VVMC_ACCObjDist_m) -> [VVMC_ACCObjDist_m]  "VVMC_ACCObjDist_m"
  VMC_FCM1/10(VVMC_ADASDBSReq_enum) -> [VVMC_ADASDBSReq_enum]  "VVMC_ADASDBSReq_enum"
  VMC_FCM1/8(VVMC_AEBVehHoldReq_flg) -> [VVMC_AEBVehHoldReq_flg]  "VVMC_AEBVehHoldReq_flg"
  VMC_FCM1/7(VVMC_ADASFaultSta_flg) -> [VVMC_ADASFaultSta_flg]  "VVMC_ADASFaultSta_flg"
  VMC_FCM1/6(VVMC_ADASAEBReq_enum) -> [VVMC_ADASAEBReq_enum]  "VVMC_ADASAEBReq_enum"
  VMC_FCM1/5(VVMC_LKATOIAct_enum) -> [VVMC_LKATOIAct_enum]  "VVMC_LKATOIAct_enum"
  VMC_FCM1/4(VVMC_LKATOIFault_flg) -> [VVMC_LKATOIFault_flg]  "VVMC_LKATOIFault_flg"
  VMC_FCM1/3(VVMC_LKAStrToqReq_Nm) -> [VVMC_LKAStrToqReq_Nm]  "VVMC_LKAStrToqReq_Nm"
  VMC_FCM1/2(VVMC_ADASLKASta_enum) -> [VVMC_ADASLKASta_enum]  "VVMC_ADASLKASta_enum"
  VMC_FCM1/1(VVMC_LateralCtrl_flg) -> [VVMC_LateralCtrl_flg]
  [VINP_ADASLanecurveR_raw32] -> VMC_FCM1/56(VINP_ADASLanecurveR_raw32)  "VINP_ADASLanecurveR_raw32"
  [VINP_ADASLanecurveL_raw32] -> VMC_FCM1/55(VINP_ADASLanecurveL_raw32)  "VINP_ADASLanecurveL_raw32"
  [VINP_ADASLanetypeL_enum] -> VMC_FCM1/54(VINP_ADASLanetypeL_enum)  "VINP_ADASLanetypeL_enum"
  [VINP_ADASLanetypeR_enum] -> VMC_FCM1/53(VINP_ADASLanetypeR_enum)  "VINP_ADASLanetypeR_enum"
  [VINP_FCMACCmode_enum] -> VMC_FCM1/52(VINP_FCMACCmode_enum)  "VINP_FCMACCmode_enum"
  [VINP_ADASLFCWarnSound_enum] -> VMC_FCM1/51(VINP_ADASLFCWarnSound_enum)  "VINP_ADASLFCWarnSound_enum"
  [VINP_LVDAACCStatusInformation_flg] -> VMC_FCM1/50(VINP_LVDAACCStatusInformation_flg)  "VINP_LVDAACCStatusInformation_flg"
  [VINP_LVDAWarning_flg] -> VMC_FCM1/49(VINP_LVDAWarning_flg)  "VINP_LVDAWarning_flg"
  [VINP_LVDAFailinfo_flg] -> VMC_FCM1/48(VINP_LVDAFailinfo_flg)  "VINP_LVDAFailinfo_flg"
  [VINP_LVDAMuteSta_enum] -> VMC_FCM1/47(VINP_LVDAMuteSta_enum)  "VINP_LVDAMuteSta_enum"
  [VINP_LVDADisabled_flg] -> VMC_FCM1/46(VINP_LVDADisabled_flg)  "VINP_LVDADisabled_flg"
  [VINP_ADASLFCHandsOffWarning_enum] -> VMC_FCM1/45(VINP_ADASLFCHandsOffWarning_enum)  "VINP_ADASLFCHandsOffWarning_enum"
  [VINP_ADASFCWMute_flg] -> VMC_FCM1/44(VINP_ADASFCWMute_flg)  "VINP_ADASFCWMute_flg"
  [VINP_ADASLDWMute_flg] -> VMC_FCM1/43(VINP_ADASLDWMute_flg)  "VINP_ADASLDWMute_flg"
  [VINP_ADASISASta_enum] -> VMC_FCM1/42(VINP_ADASISASta_enum)  "VINP_ADASISASta_enum"
  [VINP_ADASSLIFSta_enum] -> VMC_FCM1/41(VINP_ADASSLIFSta_enum)  "VINP_ADASSLIFSta_enum"
  [VINP_ADASLaneModeR_enum] -> VMC_FCM1/40(VINP_ADASLaneModeR_enum)  "VINP_ADASLaneModeR_enum"
  [VINP_ADASLaneModeL_enum] -> VMC_FCM1/39(VINP_ADASLaneModeL_enum)  "VINP_ADASLaneModeL_enum"
  [VINP_ADASLFCSta_enum] -> VMC_FCM1/38(VINP_ADASLFCSta_enum)  "VINP_ADASLFCSta_enum"
  [VINP_LKAHODSoundWarning_flg] -> VMC_FCM1/37(VINP_LKAHODSoundWarning_flg)  "VINP_LKAHODSoundWarning_flg"
  [VINP_LKAHODDisplayWarning_flg] -> VMC_FCM1/36(VINP_LKAHODDisplayWarning_flg)  "VINP_LKAHODDisplayWarning_flg"
  [VINP_ADASSLIFSpdLim_enum] -> VMC_FCM1/35(VINP_ADASSLIFSpdLim_enum)  "VINP_ADASSLIFSpdLim_enum"
  [VINP_TargetType_enum] -> VMC_FCM1/34(VINP_TargetType_enum)  "VINP_TargetType_enum"
  [VINP_ADASCAMSpdLim_enum] -> VMC_FCM1/33(VINP_ADASCAMSpdLim_enum)  "VINP_ADASCAMSpdLim_enum"
  [VINP_ADASWarningMsg_enum] -> VMC_FCM1/32(VINP_ADASWarningMsg_enum)  "VINP_ADASWarningMsg_enum"
  [VINP_ACCTakeoverReq_flg] -> VMC_FCM1/31(VINP_ACCTakeoverReq_flg)  "VINP_ACCTakeoverReq_flg"
  [VINP_ForceLowBeam_enum] -> VMC_FCM1/30(VINP_ForceLowBeam_enum)  "VINP_ForceLowBeam_enum"
  [VINP_ACCObjDstLvl_enum] -> VMC_FCM1/29(VINP_ACCObjDstLvl_enum)  "VINP_ACCObjDstLvl_enum"
  [VINP_ADASFltWrnReq_flg] -> VMC_FCM1/28(VINP_ADASFltWrnReq_flg)  "VINP_ADASFltWrnReq_flg"
  [VINP_ADASLDWSta_enum] -> VMC_FCM1/27(VINP_ADASLDWSta_enum)  "VINP_ADASLDWSta_enum"
  [VINP_ADASFCWSta_enum] -> VMC_FCM1/26(VINP_ADASFCWSta_enum)  "VINP_ADASFCWSta_enum"
  [VINP_LeftTurnLightReq_flg] -> VMC_FCM1/25(VINP_LeftTurnLightReq_flg)  "VINP_LeftTurnLightReq_flg"
  [VINP_RightTurnLightReq_flg] -> VMC_FCM1/24(VINP_RightTurnLightReq_flg)  "VINP_RightTurnLightReq_flg"
  [VINP_HazardWarningReq_flg] -> VMC_FCM1/23(VINP_HazardWarningReq_flg)  "VINP_HazardWarningReq_flg"
  [VINP_ADASForceIdle_flg] -> VMC_FCM1/22(VINP_ADASForceIdle_flg)  "VINP_ADASForceIdle_flg"
  [VINP_ADASShftPosnReq_enum] -> VMC_FCM1/21(VINP_ADASShftPosnReq_enum)  "VINP_ADASShftPosnReq_enum"
  [VINP_ADASShftPosnReqA_flg] -> VMC_FCM1/20(VINP_ADASShftPosnReqA_flg)  "VINP_ADASShftPosnReqA_flg"
  [VINP_ADASVehSpdLim_raw32] -> VMC_FCM1/19(VINP_ADASVehSpdLim_raw32)  "VINP_ADASVehSpdLim_raw32"
  [VINP_ACCComfortBandLower_mps2] -> VMC_FCM1/18(VINP_ACCComfortBandLower_mps2)  "VINP_ACCComfortBandLower_mps2"
  [VINP_ACCJerkLowerLimit_mps3] -> VMC_FCM1/17(VINP_ACCJerkLowerLimit_mps3)  "VINP_ACCJerkLowerLimit_mps3"
  [VINP_ACCComfortBandUpper_mps2] -> VMC_FCM1/16(VINP_ACCComfortBandUpper_mps2)  "VINP_ACCComfortBandUpper_mps2"
  [VINP_ACCJerkUpperLimit_mps3] -> VMC_FCM1/15(VINP_ACCJerkUpperLimit_mps3)  "VINP_ACCJerkUpperLimit_mps3"
  [VINP_ACCObjDist_m] -> VMC_FCM1/12(VINP_ACCObjDist_m)  "VINP_ACCObjDist_m"
  [VINP_ACCObjRelSpd_mps] -> VMC_FCM1/13(VINP_ACCObjRelSpd_mps)  "VINP_ACCObjRelSpd_mps"
  [VINP_TimeGapLevel_enum] -> VMC_FCM1/14(VINP_TimeGapLevel_enum)  "VINP_TimeGapLevel_enum"
  VINP_ADASLanecurveR_raw32/1 -> [VINP_ADASLanecurveR_raw32]
  VINP_ADASLanecurveL_raw32/1 -> [VINP_ADASLanecurveL_raw32]
  VINP_ADASLanetypeL_enum/1 -> [VINP_ADASLanetypeL_enum]
  VINP_ADASLanetypeR_enum/1 -> [VINP_ADASLanetypeR_enum]
  VINP_FCMACCmode_enum/1 -> [VINP_FCMACCmode_enum]
  VINP_ADASLFCWarnSound_enum/1 -> [VINP_ADASLFCWarnSound_enum]
  VINP_LVDAACCStatusInformation_flg/1 -> [VINP_LVDAACCStatusInformation_flg]
  VINP_LVDAWarning_flg/1 -> [VINP_LVDAWarning_flg]
  VINP_LVDAFailinfo_flg/1 -> [VINP_LVDAFailinfo_flg]
  VINP_LVDAMuteSta_enum/1 -> [VINP_LVDAMuteSta_enum]
  VINP_LVDADisabled_flg/1 -> [VINP_LVDADisabled_flg]
  VINP_ADASLFCHandsOffWarning_enum/1 -> [VINP_ADASLFCHandsOffWarning_enum]
  VINP_ADASFCWMute_flg/1 -> [VINP_ADASFCWMute_flg]
  VINP_ADASLDWMute_flg/1 -> [VINP_ADASLDWMute_flg]
  VINP_ADASISASta_enum/1 -> [VINP_ADASISASta_enum]
  VINP_ADASSLIFSta_enum/1 -> [VINP_ADASSLIFSta_enum]
  VINP_ADASLaneModeR_enum/1 -> [VINP_ADASLaneModeR_enum]
  VINP_ADASLaneModeL_enum/1 -> [VINP_ADASLaneModeL_enum]
  VINP_ADASLFCSta_enum/1 -> [VINP_ADASLFCSta_enum]
  VINP_LKAHODSoundWarning_flg/1 -> [VINP_LKAHODSoundWarning_flg]
  VINP_LKAHODDisplayWarning_flg/1 -> [VINP_LKAHODDisplayWarning_flg]
  VINP_ADASSLIFSpdLim_enum/1 -> [VINP_ADASSLIFSpdLim_enum]
  VINP_TargetType_enum/1 -> [VINP_TargetType_enum]
  VINP_ADASCAMSpdLim_enum/1 -> [VINP_ADASCAMSpdLim_enum]
  VINP_ADASWarningMsg_enum/1 -> [VINP_ADASWarningMsg_enum]
  VINP_ACCTakeoverReq_flg/1 -> [VINP_ACCTakeoverReq_flg]
  VINP_ForceLowBeam_enum/1 -> [VINP_ForceLowBeam_enum]
  VINP_ACCObjDstLvl_enum/1 -> [VINP_ACCObjDstLvl_enum]
  VINP_ADASFltWrnReq_flg/1 -> [VINP_ADASFltWrnReq_flg]
  VINP_ADASLDWSta_enum/1 -> [VINP_ADASLDWSta_enum]
  VINP_ADASFCWSta_enum/1 -> [VINP_ADASFCWSta_enum]
  VINP_LeftTurnLightReq_flg/1 -> [VINP_LeftTurnLightReq_flg]
  VINP_RightTurnLightReq_flg/1 -> [VINP_RightTurnLightReq_flg]
  VINP_HazardWarningReq_flg/1 -> [VINP_HazardWarningReq_flg]
  VINP_ADASForceIdle_flg/1 -> [VINP_ADASForceIdle_flg]
  VINP_ADASShftPosnReq_enum/1 -> [VINP_ADASShftPosnReq_enum]
  VINP_ADASShftPosnReqA_flg/1 -> [VINP_ADASShftPosnReqA_flg]
  VINP_ADASVehSpdLim_raw32/1 -> [VINP_ADASVehSpdLim_raw32]
  VINP_ACCComfortBandLower_mps2/1 -> [VINP_ACCComfortBandLower_mps2]
  VINP_ACCJerkLowerLimit_mps3/1 -> [VINP_ACCJerkLowerLimit_mps3]
  VINP_ACCComfortBandUpper_mps2/1 -> [VINP_ACCComfortBandUpper_mps2]
  VINP_ACCJerkUpperLimit_mps3/1 -> [VINP_ACCJerkUpperLimit_mps3]
  [Trigger_10ms_1] -> SpeedCalculation/Trigger
  ACC_Function/7(VVMC_AccPedalOvrdDISC_flg) -> [VVMC_AccPedalOvrdDISC_flg]
  [VVMC_LongAcc_Gps] -> SPD2ACC/11(VVMC_LongAcc_Gps)
  [VTQR_RrTMTqReq_Nm] -> ACC_Function/23(VTQR_RrTMTqReq_Nm)
  VTQR_RrTMTqReq_Nm/1 -> [VTQR_RrTMTqReq_Nm]
  [Trigger_10ms_2] -> SafetyControl/Trigger
  [VTQD_GearActualPosn_enum] -> CruiseControlFunction/15(VTQD_GearActualPosn_enum)
  ACC_Function/6(VVMC_ADASNegReq_flg) -> [VVMC_ADASNegReq_flg]
  VINP_RearAxlTrqReqBrk_Nm/1 -> [VINP_RearAxlTrqReqBrk_Nm]
  VINP_FrntAxlTrqReqBrk_Nm/1 -> [VINP_FrntAxlTrqReqBrk_Nm]
  [VTQD_SWC2ResUpSta_flg] -> ACC_Function/20(VTQD_SWC2ResUpSta_flg)
  [VINP_FrntAxlTrqReqBrk_Nm] -> ACC_Function/21(VINP_FrntAxlTrqReqBrk_Nm)  "VINP_FrntAxlTrqReqBrk_Nm"
  [VINP_RearAxlTrqReqBrk_Nm] -> ACC_Function/22(VINP_RearAxlTrqReqBrk_Nm)  "VINP_RearAxlTrqReqBrk_Nm"
  Constant26/1 -> Long Acceleration Calculation/4(task_time_s)
  VINP_ADASFaultSta_flg/1 -> [VINP_ADASFaultSta_flg]
  VINP_ADASAEBReq_enum/1 -> [VINP_ADASAEBReq_enum]
  VTQD_SpdCtrlSta_flg/1 -> [VTQD_SpdCtrlSta_flg]
  VINP_ADASLKASta_enum/1 -> [VINP_ADASLKASta_enum]
  VTQD_SWC2SetdownSta_flg/1 -> [VTQD_SWC2SetdownSta_flg]
  VINP_RFRawWhlSpeedV_flg/1 -> [VINP_RFRawWhlSpeedV_flg]
  VINP_ADASDBSReq_enum/1 -> [VINP_ADASDBSReq_enum]
  VINP_GRADE_Deg/1 -> [VINP_GRADE_Deg]
  VINP_LatAccelV_flg/1 -> [VINP_LatAccelV_flg]
  VINP_LFRawWhlSpeed_kph/1 -> [VINP_LFRawWhlSpeed_kph]
  VINP_RRRawWhlSpeedV_flg/1 -> [VINP_RRRawWhlSpeedV_flg]
  VINP_EPBSta_enum/1 -> [VINP_EPBSta_enum]
  VINP_VehSpeed_kph/1 -> [VINP_VehSpeed_kph]
  VINP_RFRawWhlSpeed_kph/1 -> [VINP_RFRawWhlSpeed_kph]
  VINP_BrakeSWGPIO_flg/1 -> [VINP_BrakeSWGPIO_flg]
  VINP_BrkSwSta_flg/1 -> [VINP_BrkSwSta_flg]
  VINP_ACCVehHoldReq_flg/1 -> [VINP_ACCVehHoldReq_flg]
  VINP_ACCObjDist_m/1 -> [VINP_ACCObjDist_m]
  VINP_ACCObjRelSpd_mps/1 -> [VINP_ACCObjRelSpd_mps]
  VINP_LKATOIAct_enum/1 -> [VINP_LKATOIAct_enum]
  VINP_LKATOIFault_flg/1 -> [VINP_LKATOIFault_flg]
  VINP_AEBVehHoldReq_flg/1 -> [VINP_AEBVehHoldReq_flg]
  VINP_MeterIndVehSpeed_kph/1 -> [VINP_MeterIndVehSpeed_kph]
  VINP_AEBAvail_flg/1 -> [VINP_AEBAvail_flg]
  VINP_TimeGapLevel_enum/1 -> [VINP_TimeGapLevel_enum]
  VINP_ESCOFFStatus_enum/1 -> [VINP_ESCOFFStatus_enum]
  VTQD_SWC2CANCELSta_flg/1 -> [VTQD_SWC2CANCELSta_flg]
  VINP_LFRawWhlSpeedV_flg/1 -> [VINP_LFRawWhlSpeedV_flg]
  VINP_RRRawWhlSpeed_kph/1 -> [VINP_RRRawWhlSpeed_kph]
  VINP_ACCAvail_flg/1 -> [VINP_ACCAvail_flg]
  VTQD_SWC2ResUpSta_flg/1 -> [VTQD_SWC2ResUpSta_flg]
  VINP_LRRawWhlSpeed_kph/1 -> [VINP_LRRawWhlSpeed_kph]
  VINP_LatAccel_Gps/1 -> [VINP_LatAccel_Gps]
  VINP_ADASACCSta_enum/1 -> [VINP_ADASACCSta_enum]
  VINP_ACCRequiredAccel_mps2/1 -> [VINP_ACCRequiredAccel_mps2]
  VINP_LKAStrToqReq_Nm/1 -> [VINP_LKAStrToqReq_Nm]
  VTQD_SpdCtrlMode_enum/1 -> [VTQD_SpdCtrlMode_enum]
  VINP_LRRawWhlSpeedV_flg/1 -> [VINP_LRRawWhlSpeedV_flg]
  VTQD_SetSpd_kph/1 -> [VTQD_SetSpd_kph]
  VINP_LongAccel_Gps/1 -> [VINP_LongAccel_Gps]
  VINP_ADASAEBSta_enum/1 -> [VINP_ADASAEBSta_enum]
  APP_SpdLimit_flg/1 -> [APP_SpdLimit_flg]
  APP_SpdLimit/1 -> [APP_SpdLimit]
  VINP_APSSpeedCMD_kph/1 -> [VINP_APSSpeedCMD_kph]
  VBCM_DrDoorSW_flg/1 -> [VBCM_DrDoorSW_flg]
  VDSC_DISCTurn_flg/1 -> [VDSC_DISCTurn_flg]
  VDSC_DISCSta_enum/1 -> [VDSC_DISCSta_enum]
  VDSC_DISCTargetSpd_kph/1 -> [VDSC_DISCTargetSpd_kph]
  VTQD_DriverWhlTqDem_Nm/1 -> [VTQD_DriverWhlTqDem_Nm]
  VTQD_CoordWhlTqDemFr_Nm/1 -> [VTQD_CoordWhlTqDemFr_Nm]
  VTQD_CoordWhlTqDemRr_Nm/1 -> [VTQD_CoordWhlTqDemRr_Nm]
  VTQD_LowIdleAccPedal_flg/1 -> [VTQD_LowIdleAccPedal_flg]
  VTQD_ExtShftAllow_flg/1 -> [VTQD_ExtShftAllow_flg]
  VTQD_GearActualPosn_enum/1 -> [VTQD_GearActualPosn_enum]
  VTQD_ExternalTqAllow_flg/1 -> [VTQD_ExternalTqAllow_flg]
  VINP_DriverSeatBeltCmd_flg/1 -> [VINP_DriverSeatBeltCmd_flg]
  task_time_s/1 -> [task_time_s]  "task_time_s"
  [VVMC_APSShiftPosnReq_enum] -> VVMC_APSShiftPosnReq_enum/1
  [VVMC_AEBVehHoldReq_flg] -> VVMC_AEBVehHoldReq_flg/1
  [VVMC_APSCtrlAvail_flg] -> VVMC_APSCtrlAvail_flg/1
  [VVMC_ADASActive_flg] -> VVMC_ADASActive_flg/1
  [VVMC_APSActive_flg] -> VVMC_APSActive_flg/1
  [VVMC_FeatSetSpdFinal_raw32] -> VVMC_FeatSetSpdFinal_raw32/1
  [VVMC_ACCCtrlAvail_flg] -> VVMC_ACCCtrlAvail_flg/1
  [VVMC_APSSpeedCMD_kph] -> VVMC_APSSpeedCMD_kph/1
  SPD2ACC/6(VVMC_ISOAccLimit_mps2) -> [VVMC_ISOAccLimit_mps2]
  [VVMC_VMCACCCtrlAvail_flg] -> SpeedArbitration/3(VVMC_VMCACCCtrlAvail_flg)
  FeatureSetSpeed/2(VVMC_FeatSetSpdForCalcu_kph) -> [VVMC_FeatSetSpdForCalcu_kph]
  [VVMC_FeatArbitrFinal_enum] -> ACC_Function/9(VVMC_FeatArbitrFinal_enum)
  CruiseControlFunction/5(VVMC_CCPedalOvrd_flg) -> [VVMC_CCPedalOvrd_flg]
  SPD2ACC/5(VVMC_AccCalcuPID_mps2) -> [VVMC_AccCalcuPID_mps2]
  [VVMC_CCCtrlSta_enum] -> SpeedArbitration/9(VVMC_CCCtrlSta_enum)  "VVMC_CCCtrlSta_enum"
  [VDSC_DISCTurn_flg] -> Switch5/3
  [VTQD_SWC2CANCELSta_flg] -> MSA function/4(VTQD_SWC2CANCELSta_flg)  "VTQD_SWC2CANCELSta_flg"
  MSA function/2(VVMC_MSAWhlTqReq_Nm) -> [VVMC_MSAWhlTqReq_Nm]
  [VVMC_VMCAEBCtrlAvail_flg] -> SpeedArbitration/4(VVMC_VMCAEBCtrlAvail_flg)
  [VVMC_ACCCtrlAllow_flg] -> PreConditionCheck/10(VVMC_ACCCtrlAllow_flg)  "VVMC_ACCCtrlAllow_flg"
  [VVMC_JerkPCT_pct] -> SPD2ACC/5(VVMC_JerkPCT_pct)
  SPD2ACC/7(VVMC_ISODecLimit_mps2) -> [VVMC_ISODecLimit_mps2]
  PreConditionCheck/3(VVMC_VMCCCCtrlAvail_flg) -> [VVMC_VMCCCCtrlAvail_flg]
  [VTQD_LowIdleAccPedal_flg] -> CruiseControlFunction/3(VTQD_LowIdleAccPedal_flg)  "VTQD_LowIdleAccPedal_flg"
  [VINP_ADASLKASta_enum] -> VMC_FCM1/2(VINP_ADASLKASta_enum)  "VINP_ADASLKASta_enum"
  [VTQD_ExternalTqAllow_flg] -> CruiseControlFunction/1(VTQD_ExternalTqAllow_flg)  "VTQD_ExternalTqAllow_flg"
  [VVMC_CCSpdWar_flg] -> Logical Operator/1
  [VVMC_FeatSetSpdForCalcu_kph] -> MSA function/7(VVMC_FeatSetSpdForCalcu_kph)
  Switch2/1 -> SpeedArbitration/11(VDSC_DISCTargetSpd_kph)  "VDSC_DISCTargetSpd_kph"
  [VTQD_DriverWhlTqDem_Nm] -> CruiseControlFunction/2(VTQD_DriverWhlTqDem_Nm)  "VTQD_DriverWhlTqDem_Nm"
  [VTQD_SWC1ResUpSta_flg] -> CruiseControlFunction/5(VTQD_SWC1ResUpSta_flg)  "VTQD_SWC1ResUpSta_flg"
  [VVMC_LongAcc_Gps] -> MSA function/6(VVMC_LongAcc_Gps)
  [VVMC_FeatArbitrFinal_enum] -> MSA function/8(VVMC_FeatArbitrFinal_enum)
  MSA function/1(VVMC_MSACtrlSta_enum) -> [VVMC_MSACtrlSta_enum]
  ACC_Function/2(VVMC_ACCPedalOvrd_flg) -> [VVMC_ACCPedalOvrd_flg]
  [VINP_LKATOIFault_flg] -> VMC_FCM1/4(VINP_LKATOIFault_flg)  "VINP_LKATOIFault_flg"
  SPD2ACC/4(VVMC_SPD2ACCAct_flg) -> [VVMC_SPD2ACCAct_flg]
  SPD2ACC/8(VVMC_ISOJerkLimit_mps3) -> [VVMC_ISOJerkLimit_mps3]
  [VVMC_MeterIndSpeedForCalcu_kph] -> ACC_Function/13(VVMC_MeterIndSpeedForCalcu_kph)
  [VVMC_FeatSetSpdForCalcu_kph] -> ACC_Function/11(VVMC_FeatSetSpdForCalcu_kph)
  [VTQD_SWC2ResUpSta_flg] -> MSA function/9(VTQD_SWC2ResUpSta_flg)  "VTQD_SWC2ResUpSta_flg"
  [VINP_ESCOFFStatus_enum] -> PreConditionCheck/7(VINP_ESCOFFStatus_enum)  "VINP_ESCOFFStatus_enum"
  [APP_SpdLimit] -> FeatureSetSpeed/3(APP_SpdLimit)  "APP_SpdLimit"
  [VINP_LongAccel_Gps] -> Long Acceleration Calculation/2(VINP_LongAccel_Gps)  "VINP_LongAccel_Gps"
  Cast To Single31/1 -> SpeedArbitration/7(VDSC_DISCSta_enum)  "VDSC_DISCSta_enum"
  [VTQD_SWC2SetdownSta_flg] -> MSA function/10(VTQD_SWC2SetdownSta_flg)  "VTQD_SWC2SetdownSta_flg"
  [VTQD_SWC1SetdownSta_flg] -> CruiseControlFunction/6(VTQD_SWC1SetdownSta_flg)  "VTQD_SWC1SetdownSta_flg"
  [VVMC_VMCCCCtrlAvail_flg] -> SpeedArbitration/1(VVMC_VMCCCCtrlAvail_flg)
  [VVMC_LimitPCT_pct] -> SPD2ACC/4(VVMC_LimitPCT_pct)
  SpeedArbitration/2(VVMC_FeatReqSpd_kph) -> [VVMC_FeatReqSpd_kph]
  [VVMC_FeatArbitrFinal_enum] -> CruiseControlFunction/13(VVMC_FeatArbitrFinal_enum)
  [VVMC_VehicleSpeed_kph] -> CruiseControlFunction/10(VVMC_VehicleSpeed_kph)
  [VINP_ADASAEBSta_enum] -> Cast To Single7/1
  [VTQD_SpdCtrlMode_enum] -> MSA function/3(<VTQD_SpdCtrlMode_enum>)  "VTQD_SpdCtrlMode_enum"
  [VINP_AEBAvail_flg] -> PreConditionCheck/6(VINP_AEBAvail_flg)  "VINP_AEBAvail_flg"
  [VVMC_LongAcc_Gps] -> ACC_Function/8(VVMC_LongAcc_Gps)
  [VBCM_DrDoorSW_flg] -> PreConditionCheck/2(VBCM_DrDoorSW_flg)  "VBCM_DrDoorSW_flg"
  ACC_Function/5(VVMC_TimeGapCalcu_s) -> [VVMC_TimeGapCalcu_s]
  [VINP_ADASAEBReq_enum] -> SpeedArbitration/5(VINP_ADASAEBReq_enum)  "VINP_ADASAEBReq_enum"
  Cast To Single7/1 -> CruiseControlFunction/14(VINP_ADASAEBSta_enum)  "VINP_ADASAEBSta_enum"
  [VTQD_CoordWhlTqDemRr_Nm] -> ACC_Function/5(VTQD_CoordWhlTqDemRr_Nm)  "VTQD_CoordWhlTqDemRr_Nm"
  [VINP_GRADE_Deg] -> Long Acceleration Calculation/1(VINP_GRADE_Deg)  "VINP_GRADE_Deg"
  Cast To Single34/1 -> SpeedArbitration/13(VDSC_DISCTurn_flg)  "VDSC_DISCTurn_flg"
  Cast To Single33/1 -> SpeedArbitration/6(VINP_ADASAEBSta_enum)  "VINP_ADASAEBSta_enum"
  [VTQD_SWC1CANCELSta_flg] -> CruiseControlFunction/7(VTQD_SWC1CANCELSta_flg)  "VTQD_SWC1CANCELSta_flg"
  [VINP_BrakeSWGPIO_flg] -> CruiseControlFunction/8(VINP_BrakeSWGPIO_flg)  "VINP_BrakeSWGPIO_flg"
  PreConditionCheck/1(VVMC_VMCACCCtrlAvail_flg) -> [VVMC_VMCACCCtrlAvail_flg]
  [VVMC_VehicleSpeed_kph] -> MSA function/5(VVMC_VehicleSpeed_kph)
  [VINP_ADASFaultSta_flg] -> VMC_FCM1/7(VINP_ADASFaultSta_flg)  "VINP_ADASFaultSta_flg"
  [VINP_BrkSwSta_flg] -> CruiseControlFunction/9(VINP_BrkSwSta_flg)  "VINP_BrkSwSta_flg"
  [VTQD_ExternalTqAllow_flg] -> MSA function/1(VTQD_ExternalTqAllow_flg)  "VTQD_ExternalTqAllow_flg"
  CruiseControlFunction/3(VVMC_CruzWhlTqReq_Nm) -> [VVMC_CruzWhlTqReq_Nm]
  Long Acceleration Calculation/1(VVMC_LongAcc_Gps) -> [VVMC_LongAcc_Gps]
  [VVMC_MSASpdWar_flg] -> Logical Operator/2
  [VTQD_LowIdleAccPedal_flg] -> ACC_Function/6(VTQD_LowIdleAccPedal_flg)  "VTQD_LowIdleAccPedal_flg"
  SpeedArbitration/1(VVMC_FeatArbitrSta_enum) -> [VVMC_FeatArbitrSta_enum]
  [VINP_EPBSta_enum] -> PreConditionCheck/4(VINP_EPBSta_enum)  "VINP_EPBSta_enum"
  [VINP_ADASACCSta_enum] -> VMC_FCM1/11(VINP_ADASACCSta_enum)  "VINP_ADASACCSta_enum"
  [VVMC_FeatSetSpdForCalcu_kph] -> SpeedArbitration/12(VVMC_FeatSetSpdForCalcu_kph)
  [VTQD_DriverWhlTqDem_Nm] -> ACC_Function/2(VTQD_DriverWhlTqDem_Nm)  "VTQD_DriverWhlTqDem_Nm"
  [VVMC_FeatArbitrFinal_enum] -> VMC_FCM1/1(VVMC_FeatArbitrFinal_enum)
  [VINP_LKAStrToqReq_Nm] -> VMC_FCM1/3(VINP_LKAStrToqReq_Nm)  "VINP_LKAStrToqReq_Nm"
  [VINP_AEBVehHoldReq_flg] -> VMC_FCM1/8(VINP_AEBVehHoldReq_flg)  "VINP_AEBVehHoldReq_flg"
  [VVMC_FeatArbitrSta_enum] -> SPD2ACC/1(VVMC_FeatArbitrSta_enum)
  [VINP_ACCVehHoldReq_flg] -> VMC_FCM1/9(VINP_ACCVehHoldReq_flg)  "VINP_ACCVehHoldReq_flg"
  [VINP_ADASAEBReq_enum] -> VMC_FCM1/6(VINP_ADASAEBReq_enum)  "VINP_ADASAEBReq_enum"
  [VDSC_DISCSta_enum] -> Switch4/3
  SPD2ACC/2(VVMC_DISCReqAcc_mps2) -> [VVMC_DISCReqAcc_mps2]  "VVMC_DISCReqAcc_mps2"
  [VINP_ACCRequiredAccel_mps2] -> SPD2ACC/9(VINP_ACCRequiredAccel_mps2)  "VINP_ACCRequiredAccel_mps2"
  [VINP_ADASACCSta_enum] -> SPD2ACC/2(VINP_ADASACCSta_enum)  "VINP_ADASACCSta_enum"
  [VVMC_MeterIndSpeedForCalcu_kph] -> SPD2ACC/7(VVMC_MeterIndSpeedForCalcu_kph)
  [VTQD_SpdCtrlMode_enum] -> CruiseControlFunction/4(<VTQD_SpdCtrlMode_enum>)  "VTQD_SpdCtrlMode_enum"
  SPD2ACC/1(VVMC_ACCRequiredAccel_mps2) -> [VVMC_ACCRequiredAccel_mps2]
  [VINP_ACCAvail_flg] -> PreConditionCheck/5(VINP_ACCAvail_flg)  "VINP_ACCAvail_flg"
  FeatureSetSpeed/1(VVMC_FeatSetSpdFinal_raw32) -> [VVMC_FeatSetSpdFinal_raw32]
  PreConditionCheck/2(VVMC_VMCAEBCtrlAvail_flg) -> [VVMC_VMCAEBCtrlAvail_flg]
  [VINP_APSStaSystem_enum] -> PreConditionCheck/8(VINP_APSStaSystem_enum)  "VINP_APSStaSystem_enum"
  [APP_SpdLimit_flg] -> FeatureSetSpeed/1(APP_SpdLimit_flg)  "APP_SpdLimit_flg"
  [VTQD_ExternalTqAllow_flg] -> PreConditionCheck/9(VTQD_ExternalTqAllow_flg)  "VTQD_ExternalTqAllow_flg"
  [VINP_ADASAEBSta_enum] -> Cast To Single33/1
  ACC_Function/4(VVMC_ADASActive_flg) -> [VVMC_ADASActive_flg]
  [VVMC_LongAcc_Gps] -> CruiseControlFunction/11(VVMC_LongAcc_Gps)
  [VVMC_ActACCRequiredAccel_mps2] -> ACC_Function/10(VVMC_ActACCRequiredAccel_mps2)
  Logical Operator/1 -> [VVMC_CCMSASpdWar_flg]  "VVMC_CCMSASpdWar_flg"
  [VTQD_DriverWhlTqDem_Nm] -> MSA function/2(VTQD_DriverWhlTqDem_Nm)  "VTQD_DriverWhlTqDem_Nm"
  MSA function/4(VVMC_MSAActive_flg) -> [VVMC_MSAActive_flg]
  ACC_Function/1(VVMC_ACCCtrlAvail_flg) -> [VVMC_ACCCtrlAvail_flg]
  CruiseControlFunction/1(VVMC_CCCtrlSta_enum) -> [VVMC_CCCtrlSta_enum]
  [VINP_ADASDBSReq_enum] -> VMC_FCM1/10(VINP_ADASDBSReq_enum)  "VINP_ADASDBSReq_enum"
  [VVMC_SafetyCtrl_flg] -> SPD2ACC/8(VVMC_SafetyCtrl_flg)  "VVMC_SafetyCtrl_flg"
  [VTQD_GearActualPosn_enum] -> PreConditionCheck/3(VTQD_GearActualPosn_enum)  "VTQD_GearActualPosn_enum"
  PreConditionCheck/4(VVMC_VMCMSACtrlAvail_flg) -> [VVMC_VMCMSACtrlAvail_flg]
  MSA function/3(VVMC_MSASpdWar_flg) -> [VVMC_MSASpdWar_flg]
  [VTQD_SetSpd_kph] -> FeatureSetSpeed/4(VTQD_SetSpd_kph)  "VTQD_SetSpd_kph"
  SpeedCalculation/1(VVMC_MeterIndSpeed_raw32) -> [VVMC_MeterIndSpeed_raw32]
  [VINP_DriverSeatBeltCmd_flg] -> PreConditionCheck/1(VINP_DriverSeatBeltCmd_flg)  "VINP_DriverSeatBeltCmd_flg"
  [VVMC_MSACtrlSta_enum] -> SpeedArbitration/10(VVMC_MSACtrlSta_enum)  "VVMC_MSACtrlSta_enum"
  [VVMC_FeatSetSpdForCalcu_kph] -> CruiseControlFunction/12(VVMC_FeatSetSpdForCalcu_kph)
  [VINP_LKATOIAct_enum] -> VMC_FCM1/5(VINP_LKATOIAct_enum)  "VINP_LKATOIAct_enum"
  [VTQD_SpdCtrlSta_flg] -> FeatureSetSpeed/2(VTQD_SpdCtrlSta_flg)  "VTQD_SpdCtrlSta_flg"
  CruiseControlFunction/2(VVMC_CCSpdWar_flg) -> [VVMC_CCSpdWar_flg]
  CruiseControlFunction/4(VVMC_CruzActive_flg) -> [VVMC_CruzActive_flg]
  [VVMC_FeatReqSpd_kph] -> SPD2ACC/3(VVMC_FeatReqSpd_kph)
  [VINP_TimeGapLevel_enum] -> ACC_Function/14(VINP_TimeGapLevel_enum)  "VINP_TimeGapLevel_enum"
  [VVMC_VMCMSACtrlAvail_flg] -> SpeedArbitration/2(VVMC_VMCMSACtrlAvail_flg)
  SpeedArbitration/3(VVMC_JerkPCT_pct) -> [VVMC_JerkPCT_pct]
  [VVMC_VehicleSpeed_kph] -> ACC_Function/7(VVMC_VehicleSpeed_kph)
  [VTQD_ExternalTqAllow_flg] -> ACC_Function/3(VTQD_ExternalTqAllow_flg)  "VTQD_ExternalTqAllow_flg"
  SpeedArbitration/4(VVMC_LimitPCT_pct) -> [VVMC_LimitPCT_pct]
  [task_time_s] -> ACC_Function/1(task_time_s)  "task_time_s"
  [VTQD_CoordWhlTqDemFr_Nm] -> ACC_Function/4(VTQD_CoordWhlTqDemFr_Nm)  "VTQD_CoordWhlTqDemFr_Nm"
  ACC_Function/3(VVMC_ADASWhlTqReq_Nm) -> [VVMC_ADASWhlTqReq_Nm]
  [VINP_ACCObjDist_m] -> ACC_Function/12(VINP_ACCObjDist_m)  "VINP_ACCObjDist_m"
  SPD2ACC/3(VVMC_FeatArbitrFinal_enum) -> [VVMC_FeatArbitrFinal_enum]
  [VINP_ADASACCSta_enum] -> SpeedArbitration/8(VINP_ADASACCSta_enum)  "VINP_ADASACCSta_enum"
  VINP_Distanceunit_flg/1 -> [VINP_Distanceunit_flg]
  [VVMC_VehicleSpeed_kph] -> SPD2ACC/6(VVMC_VehicleSpeed_kph)
  VINP_RrTMSpdNidec_rpm/1 -> Switch3/3
  VINP_MCPressure_bar/1 -> [VINP_MCPressure_bar]
  VINP_ESCADASSta_enum/1 -> [VINP_ESCADASSta_enum]
  VTQD_RegenMode_enum/1 -> [VTQD_RegenMode_enum]
  VINP_RrRBCActive_flg/1 -> [VINP_RrRBCActive_flg]
  VINP_FrRBCActive_flg/1 -> [VINP_FrRBCActive_flg]
  [VINP_FrTMSpd_rpm] -> ACC_Function/15(VINP_FrTMSpd_rpm)  "VINP_FrTMSpd_rpm"
  [VINP_RrTMSpd_rpm] -> ACC_Function/16(VINP_RrTMSpd_rpm)  "VINP_RrTMSpd_rpm"
  [VINP_MCPressure_bar] -> ACC_Function/17(VINP_MCPressure_bar)  "VINP_MCPressure_bar"
  [VINP_ESCADASSta_enum] -> ACC_Function/18(VINP_ESCADASSta_enum)  "VINP_ESCADASSta_enum"
  [VVMC_VehicleSpeed_kph] -> Long Acceleration Calculation/3(VVMC_VehicleSpeed_kph)
  SpeedCalculation/2(VVMC_VehicleSpeed_mph) -> [VVMC_VehicleSpeed_mph]
  SpeedCalculation/3(VVMC_VehicleSpeed_kph) -> [VVMC_VehicleSpeed_kph]
  [task_time_s] -> PreConditionCheck/11(task_time_s)
  [VVMC_FeatReqSpd_kph] -> ACC_Function/19(VVMC_FeatReqSpd_kph)
  SpeedCalculation/4(VVMC_MeterIndSpeedForCalcu_kph) -> [VVMC_MeterIndSpeedForCalcu_kph]
  [task_time_s] -> SPD2ACC/10(task_time_s)
  [VVMC_FeatArbitrFinal_enum] -> initial = 0/1
  [VVMC_MeterIndSpeedForCalcu_kph] -> SpeedArbitration/14(VVMC_MeterIndSpeedForCalcu_kph)
  [VVMC_VehicleSpeed_kph] -> SpeedArbitration/15(VVMC_VehicleSpeed_kph)
  SPD2ACC/15(VVMC_ReqBrkJoin_flg) -> [VVMC_ReqBrkJoin_flg]
  [VVMC_ReqBrkJoin_flg] -> ACC_Function/53(VVMC_ReqBrkJoin_flg)
  [VVMC_MeterIndSpeed_raw32] -> CruiseControlFunction/27(VVMC_MeterIndSpeed_raw32)
  [VVMC_MeterIndSpeed_raw32] -> MSA function/30(VVMC_MeterIndSpeed_raw32)
  [VVMC_VehPitchAngleSta_enum] -> VVMC_VehPitchAngleSta_enum/1
  [Trigger_LongAccel] -> Long Acceleration Calculation/Trigger
  Scheduler1/1(Trigger_LongAccel()) -> [Trigger_LongAccel]
  ACC_Function/12(VVMC_ACCWhlTqLowerLim_Nm) -> [VVMC_ACCWhlTqLowerLim_Nm]
  [VVMC_ACCWhlTqLowerLim_Nm] -> SPD2ACC/35(VVMC_ACCWhlTqLowerLim_Nm)
  [VINP_ACCRequiredAccel_mps2] -> Long Acceleration Calculation/10(VINP_ACCRequiredAccel_mps2)
  [VINP_RrTMSpd_rpm] -> SPD2ACC/36(VINP_RrTMSpd_rpm)
  [VINP_RDCActive_enum] -> ACC_Function/54(VINP_RDCActive_enum)
  [VINP_RDCActive_enum] -> MSA function/31(VINP_RDCActive_enum)
  [VINP_RDCActive_enum] -> CruiseControlFunction/28(VINP_RDCActive_enum)
  Constant1/1 -> SpeedCalculation/7(task_time_s)
  [task_time_s] -> VMC_FCM1/62(task_time_s)
  [VINP_BrkSwSta_flg] -> ACC_Function/55(VINP_BrkSwSta_flg)
  [VINP_LFWhlRotDir_enum] -> ACC_Function/56(VINP_LFWhlRotDir_enum)
  [VINP_LRWhlRotDir_enum] -> ACC_Function/57(VINP_LRWhlRotDir_enum)
  [VINP_RFWhlRotDir_enum] -> ACC_Function/58(VINP_RFWhlRotDir_enum)
  [VINP_RRWhlRotDir_enum] -> ACC_Function/59(VINP_RRWhlRotDir_enum)
  [VINP_VehicleType_enum] -> Equal3/1
  Constant3/1 -> Equal3/2
  Equal3/1 -> Switch9/2
  VINP_FrEDURealTMTq_Nm/1 -> Switch9/1
  VINP_FrEDURealTMTqNidec_Nm/1 -> Switch9/3
  Switch9/1 -> [VINP_FrEDURealTMTq_Nm]  "VINP_FrEDURealTMTq_Nm"
  Equal4/1 -> Switch10/2
  Constant4/1 -> Equal4/2
  [VINP_VehicleType_enum] -> Equal4/1
  VINP_FrEDURotateDirction_enum/1 -> Switch10/1
  VINP_FrEDURotateDirctionNidec_enum/1 -> Switch10/3
  Switch10/1 -> [VINP_FrEDURotateDirction_enum]  "VINP_FrEDURotateDirction_enum"
  Switch11/1 -> [VINP_RrEDURealTMTq_Nm]  "VINP_RrEDURealTMTq_Nm"
  Equal5/1 -> Switch11/2
  Constant5/1 -> Equal5/2
  VINP_RrEDURealTMTq_Nm/1 -> Switch11/1
  VINP_RrEDURealTMTqNidec_Nm/1 -> Switch11/3
  [VINP_VehicleType_enum] -> Equal5/1
  Switch12/1 -> [VINP_RrEDURotateDirction_enum]  "VINP_RrEDURotateDirction_enum"
  [VINP_VehicleType_enum] -> Equal6/1
  Constant8/1 -> Equal6/2
  Equal6/1 -> Switch12/2
  VINP_RrEDURotateDirctionNidec_enum/1 -> Switch12/3
  VINP_RrEDURotateDirction_enum/1 -> Switch12/1
  [VINP_RrEDURotateDirction_enum] -> ACC_Function/63(VINP_RrEDURotateDirction_enum)
  [VINP_RrEDURealTMTq_Nm] -> ACC_Function/62(VINP_RrEDURealTMTq_Nm)
  [VINP_FrEDURotateDirction_enum] -> ACC_Function/61(VINP_FrEDURotateDirction_enum)
  [VINP_FrEDURealTMTq_Nm] -> ACC_Function/60(VINP_FrEDURealTMTq_Nm)
  ACC_Function/13(VVMC_RrWhlStandstill_flg) -> [VVMC_RrWhlStandstill_flg]
  [VVMC_RrWhlStandstill_flg] -> SPD2ACC/37(VVMC_RrWhlStandstill_flg)
  [VINP_DMSStatus_enum] -> VMC_FCM1/63(VINP_DMSStatus_enum)
  [VINP_DMSWarningFatigue_enum] -> VMC_FCM1/64(VINP_DMSWarningFatigue_enum)
  [VINP_DMSWarningUnresponsive_flg] -> VMC_FCM1/65(VINP_DMSWarningUnresponsive_flg)
  VINP_DMSWarningUnresponsive_flg/1 -> [VINP_DMSWarningUnresponsive_flg]
  VINP_DMSWarningFatigue_enum/1 -> [VINP_DMSWarningFatigue_enum]
  VINP_DMSStatus_enum/1 -> [VINP_DMSStatus_enum]
  [VVMC_ACCVehHoldReq_flg] -> ACC_Function/64(VVMC_ACCVehHoldReq_flg)
  [VINP_TimeGapLevel_enum] -> SPD2ACC/38(VINP_TimeGapLevel_enum)
  VINP_LongAccelV_flg/1 -> [VINP_LongAccelV_flg]
  [VINP_RrRBCActive_flg] -> Terminator/1
  [VINP_FrRBCActive_flg] -> Terminator1/1
  SafetyControl/15(VVMC_LongAccelCalcuRrWhlRaw_gps) -> [VVMC_LongAccelCalcuRrWhlRaw_gps]
  SafetyControl/14(VVMC_LongAccelCalcuFrWhlRaw_gps) -> [VVMC_LongAccelCalcuFrWhlRaw_gps]
  [VVMC_LongAccelCalcuFrWhlRaw_gps] -> Long Acceleration Calculation/11(VVMC_LongAccelCalcuFrWhlRaw_gps)
  [VVMC_LongAccelCalcuRrWhlRaw_gps] -> Long Acceleration Calculation/12(VVMC_LongAccelCalcuRrWhlRaw_gps)
  Long Acceleration Calculation/3(VVMC_LongAccFrWhl_Gps) -> [VVMC_LongAccFrWhl_Gps]
  Long Acceleration Calculation/4(VVMC_LongAccRrWhl_Gps) -> [VVMC_LongAccRrWhl_Gps]
  [VVMC_LongAccRrWhl_Gps] -> ACC_Function/68(VVMC_LongAccRrWhl_Gps)
  [VVMC_LongAccFrWhl_Gps] -> ACC_Function/67(VVMC_LongAccFrWhl_Gps)
  SafetyControl/16(VVMC_FrWhlSpdInvalid_flg) -> [VVMC_FrWhlSpdInvalid_flg]
  SafetyControl/17(VVMC_RrWhlSpdInvalid_flg) -> [VVMC_RrWhlSpdInvalid_flg]
  [VVMC_FrWhlSpdInvalid_flg] -> ACC_Function/65(VVMC_FrWhlSpdInvalid_flg)
  [VVMC_RrWhlSpdInvalid_flg] -> ACC_Function/66(VVMC_RrWhlSpdInvalid_flg)
  [VVMC_FrWhlSpdInvalid_flg] -> Long Acceleration Calculation/13(VVMC_FrWhlSpdInvalid_flg)
  [VVMC_RrWhlSpdInvalid_flg] -> Long Acceleration Calculation/14(VVMC_RrWhlSpdInvalid_flg)
  [VVMC_CalibratedGyroY_Dps] -> Long Acceleration Calculation/15(VVMC_CalibratedGyroY_Dps)
  [VVMC_CalibratedAccX_G] -> Long Acceleration Calculation/16(VVMC_CalibratedAccX_G)
  [VVMC_CalibratedAccY_G] -> Long Acceleration Calculation/17(VVMC_CalibratedAccY_G)
  [VVMC_CalibratedAccZ_G] -> Long Acceleration Calculation/18(VVMC_CalibratedAccZ_G)
  [VINP_BrkPedalPos_pct] -> Long Acceleration Calculation/19(VINP_BrkPedalPos_pct)
  [VTQD_GearActualPosn_enum] -> Long Acceleration Calculation/20(VTQD_GearActualPosn_enum)
  [VDHP_ActAPSPosn_pct] -> Long Acceleration Calculation/21(VDHP_ActAPSPosn_pct)
  [VTQD_RegenMode_enum] -> Long Acceleration Calculation/22(VTQD_RegenMode_enum)
  [VTQD_VehActSpd_kph] -> Long Acceleration Calculation/23(VTQD_VehActSpd_kph)
  VTQD_PreLoadPreEn_flg/1 -> [VTQD_PreLoadPreEn_flg]
  [VTQD_PreLoadPreEn_flg] -> Long Acceleration Calculation/24(VTQD_PreLoadPreEn_flg)
  Long Acceleration Calculation/5(VVMC_EstSlopeCalBase_Deg) -> [VVMC_EstSlopeCalBase_Deg]
  Long Acceleration Calculation/6(VVMC_IMUEstSlope_Deg1) -> [VVMC_IMUEstSlope_Deg1]
  Long Acceleration Calculation/7(VVMC_FinalSlop_deg) -> [VVMC_FinalSlop_deg]
  [VTQR_RrTMTqReq_Nm] -> Long Acceleration Calculation/25(VTQR_RrTMTqReq_Nm)
  [VTQR_FrTMTqReq_Nm] -> Long Acceleration Calculation/26(VTQR_FrTMTqReq_Nm)
  [VPMM_DrivetrainSelect_enum] -> Long Acceleration Calculation/27(VPMM_DrivetrainSelect_enum)
